simulink model "s_deng_rev1_13_wide"  (R2016b)
(part 3 of 68)

      mask Display:
      | port_label('input', 1, 'd');
      | port_label('output', 1, 'q');
      | disp(['Z^-', num2str(latency)]);
  pipeline80 : Subsystem  AncestorBlock=casper_library_delays/pipeline  mask(pipeline){latency=1}
      mask help:
      | An explicitly laid-out delay line to avoid mapping to SRL16s
      | for use in pipelining to help achieve timing closure.
      mask init:
      | pipeline_init(gcb,'latency',latency);
      settings: AttributesFormatString=Latency = %<latency>
      mask Display:
      | port_label('input', 1, 'd');
      | port_label('output', 1, 'q');
      | disp(['Z^-', num2str(latency)]);
  pipeline81 : Subsystem  AncestorBlock=casper_library_delays/pipeline  mask(pipeline){latency=3}
      mask help:
      | An explicitly laid-out delay line to avoid mapping to SRL16s
      | for use in pipelining to help achieve timing closure.
      mask init:
      | pipeline_init(gcb,'latency',latency);
      settings: AttributesFormatString=Latency = %<latency>
      mask Display:
      | port_label('input', 1, 'd');
      | port_label('output', 1, 'q');
      | disp(['Z^-', num2str(latency)]);
  pipeline82 : Subsystem  AncestorBlock=casper_library_delays/pipeline  mask(pipeline){latency=1}
      mask help:
      | An explicitly laid-out delay line to avoid mapping to SRL16s
      | for use in pipelining to help achieve timing closure.
      mask init:
      | pipeline_init(gcb,'latency',latency);
      settings: AttributesFormatString=Latency = %<latency>
      mask Display:
      | port_label('input', 1, 'd');
      | port_label('output', 1, 'q');
      | disp(['Z^-', num2str(latency)]);
  pipeline83 : Subsystem  AncestorBlock=casper_library_delays/pipeline  mask(pipeline){latency=1}
      mask help:
      | An explicitly laid-out delay line to avoid mapping to SRL16s
      | for use in pipelining to help achieve timing closure.
      mask init:
      | pipeline_init(gcb,'latency',latency);
      settings: AttributesFormatString=Latency = %<latency>
      mask Display:
      | port_label('input', 1, 'd');
      | port_label('output', 1, 'q');
      | disp(['Z^-', num2str(latency)]);
  pipeline84 : Subsystem  AncestorBlock=casper_library_delays/pipeline  mask(pipeline){latency=1}
      mask help:
      | An explicitly laid-out delay line to avoid mapping to SRL16s
      | for use in pipelining to help achieve timing closure.
      mask init:
      | pipeline_init(gcb,'latency',latency);
      settings: AttributesFormatString=Latency = %<latency>
      mask Display:
      | port_label('input', 1, 'd');
      | port_label('output', 1, 'q');
      | disp(['Z^-', num2str(latency)]);
  pipeline85 : Subsystem  AncestorBlock=casper_library_delays/pipeline  mask(pipeline){latency=1}
      mask help:
      | An explicitly laid-out delay line to avoid mapping to SRL16s
      | for use in pipelining to help achieve timing closure.
      mask init:
      | pipeline_init(gcb,'latency',latency);
      settings: AttributesFormatString=Latency = %<latency>
      mask Display:
      | port_label('input', 1, 'd');
      | port_label('output', 1, 'q');
      | disp(['Z^-', num2str(latency)]);
  pipeline86 : Subsystem  AncestorBlock=casper_library_delays/pipeline  mask(pipeline){latency=3}
      mask help:
      | An explicitly laid-out delay line to avoid mapping to SRL16s
      | for use in pipelining to help achieve timing closure.
      mask init:
      | pipeline_init(gcb,'latency',latency);
      settings: AttributesFormatString=Latency = %<latency>
      mask Display:
      | port_label('input', 1, 'd');
      | port_label('output', 1, 'q');
      | disp(['Z^-', num2str(latency)]);
  pipeline87 : Subsystem  AncestorBlock=casper_library_delays/pipeline  mask(pipeline){latency=2}
      mask help:
      | An explicitly laid-out delay line to avoid mapping to SRL16s
      | for use in pipelining to help achieve timing closure.
      mask init:
      | pipeline_init(gcb,'latency',latency);
      settings: AttributesFormatString=Latency = %<latency>
      mask Display:
      | port_label('input', 1, 'd');
      | port_label('output', 1, 'q');
      | disp(['Z^-', num2str(latency)]);
  pipeline88 : Subsystem  AncestorBlock=casper_library_delays/pipeline  mask(pipeline){latency=2}
      mask help:
      | An explicitly laid-out delay line to avoid mapping to SRL16s
      | for use in pipelining to help achieve timing closure.
      mask init:
      | pipeline_init(gcb,'latency',latency);
      settings: AttributesFormatString=Latency = %<latency>
      mask Display:
      | port_label('input', 1, 'd');
      | port_label('output', 1, 'q');
      | disp(['Z^-', num2str(latency)]);
  pipeline89 : Subsystem  AncestorBlock=casper_library_delays/pipeline  mask(pipeline){latency=2}
      mask help:
      | An explicitly laid-out delay line to avoid mapping to SRL16s
      | for use in pipelining to help achieve timing closure.
      mask init:
      | pipeline_init(gcb,'latency',latency);
      settings: AttributesFormatString=Latency = %<latency>
      mask Display:
      | port_label('input', 1, 'd');
      | port_label('output', 1, 'q');
      | disp(['Z^-', num2str(latency)]);
  pipeline9 : Subsystem  AncestorBlock=casper_library_delays/pipeline  mask(pipeline){latency=3}
      mask help:
      | An explicitly laid-out delay line to avoid mapping to SRL16s
      | for use in pipelining to help achieve timing closure.
      mask init:
      | pipeline_init(gcb,'latency',latency);
      settings: AttributesFormatString=Latency = %<latency>
      mask Display:
      | port_label('input', 1, 'd');
      | port_label('output', 1, 'q');
      | disp(['Z^-', num2str(latency)]);
  pipeline90 : Subsystem  AncestorBlock=casper_library_delays/pipeline  mask(pipeline){latency=2}
      mask help:
      | An explicitly laid-out delay line to avoid mapping to SRL16s
      | for use in pipelining to help achieve timing closure.
      mask init:
      | pipeline_init(gcb,'latency',latency);
      settings: AttributesFormatString=Latency = %<latency>
      mask Display:
      | port_label('input', 1, 'd');
      | port_label('output', 1, 'q');
      | disp(['Z^-', num2str(latency)]);
  pipeline91 : Subsystem  AncestorBlock=casper_library_delays/pipeline  mask(pipeline){latency=2}
      mask help:
      | An explicitly laid-out delay line to avoid mapping to SRL16s
      | for use in pipelining to help achieve timing closure.
      mask init:
      | pipeline_init(gcb,'latency',latency);
      settings: AttributesFormatString=Latency = %<latency>
      mask Display:
      | port_label('input', 1, 'd');
      | port_label('output', 1, 'q');
      | disp(['Z^-', num2str(latency)]);
  pipeline92 : Subsystem  AncestorBlock=casper_library_delays/pipeline  mask(pipeline){latency=2}
      mask help:
      | An explicitly laid-out delay line to avoid mapping to SRL16s
      | for use in pipelining to help achieve timing closure.
      mask init:
      | pipeline_init(gcb,'latency',latency);
      settings: AttributesFormatString=Latency = %<latency>
      mask Display:
      | port_label('input', 1, 'd');
      | port_label('output', 1, 'q');
      | disp(['Z^-', num2str(latency)]);
  pipeline93 : Subsystem  AncestorBlock=casper_library_delays/pipeline  mask(pipeline){latency=2}
      mask help:
      | An explicitly laid-out delay line to avoid mapping to SRL16s
      | for use in pipelining to help achieve timing closure.
      mask init:
      | pipeline_init(gcb,'latency',latency);
      settings: AttributesFormatString=Latency = %<latency>
      mask Display:
      | port_label('input', 1, 'd');
      | port_label('output', 1, 'q');
      | disp(['Z^-', num2str(latency)]);
  pipeline94 : Subsystem  AncestorBlock=casper_library_delays/pipeline  mask(pipeline){latency=2}
      mask help:
      | An explicitly laid-out delay line to avoid mapping to SRL16s
      | for use in pipelining to help achieve timing closure.
      mask init:
      | pipeline_init(gcb,'latency',latency);
      settings: AttributesFormatString=Latency = %<latency>
      mask Display:
      | port_label('input', 1, 'd');
      | port_label('output', 1, 'q');
      | disp(['Z^-', num2str(latency)]);
  pipeline95 : Subsystem  AncestorBlock=casper_library_delays/pipeline  mask(pipeline){latency=2}
      mask help:
      | An explicitly laid-out delay line to avoid mapping to SRL16s
      | for use in pipelining to help achieve timing closure.
      mask init:
      | pipeline_init(gcb,'latency',latency);
      settings: AttributesFormatString=Latency = %<latency>
      mask Display:
      | port_label('input', 1, 'd');
      | port_label('output', 1, 'q');
      | disp(['Z^-', num2str(latency)]);
  pipeline96 : Subsystem  AncestorBlock=casper_library_delays/pipeline  mask(pipeline){latency=2}
      mask help:
      | An explicitly laid-out delay line to avoid mapping to SRL16s
      | for use in pipelining to help achieve timing closure.
      mask init:
      | pipeline_init(gcb,'latency',latency);
      settings: AttributesFormatString=Latency = %<latency>
      mask Display:
      | port_label('input', 1, 'd');
      | port_label('output', 1, 'q');
      | disp(['Z^-', num2str(latency)]);
  pipeline97 : Subsystem  AncestorBlock=casper_library_delays/pipeline  mask(pipeline){latency=2}
      mask help:
      | An explicitly laid-out delay line to avoid mapping to SRL16s
      | for use in pipelining to help achieve timing closure.
      mask init:
      | pipeline_init(gcb,'latency',latency);
      settings: AttributesFormatString=Latency = %<latency>
      mask Display:
      | port_label('input', 1, 'd');
      | port_label('output', 1, 'q');
      | disp(['Z^-', num2str(latency)]);
  pipeline98 : Subsystem  AncestorBlock=casper_library_delays/pipeline  mask(pipeline){latency=2}
      mask help:
      | An explicitly laid-out delay line to avoid mapping to SRL16s
      | for use in pipelining to help achieve timing closure.
      mask init:
      | pipeline_init(gcb,'latency',latency);
      settings: AttributesFormatString=Latency = %<latency>
      mask Display:
      | port_label('input', 1, 'd');
      | port_label('output', 1, 'q');
      | disp(['Z^-', num2str(latency)]);
  pipeline99 : Subsystem  AncestorBlock=casper_library_delays/pipeline  mask(pipeline){latency=2}
      mask help:
      | An explicitly laid-out delay line to avoid mapping to SRL16s
      | for use in pipelining to help achieve timing closure.
      mask init:
      | pipeline_init(gcb,'latency',latency);
      settings: AttributesFormatString=Latency = %<latency>
      mask Display:
      | port_label('input', 1, 'd');
      | port_label('output', 1, 'q');
      | disp(['Z^-', num2str(latency)]);
  pkt_rate0 : Subsystem
  pkt_size0 : Subsystem  Tag=xps:sw_reg  AncestorBlock=xps_library/software_register  mask(swreg){io_dir=From Processor, io_delay=0, sample_period=1, names=reg, bitwidths=32, bin_pts=0, arith_types=0, sim_port=on, show_format=on}
      mask prompts: io_dir "I/O direction"; io_delay "I/O delay"; sample_period "Sample period"; names "Bitfield names [msb...lsb]"; bitwidths "Bitfield widths"; bin_pts "Bitfield binary pts"; arith_types "Bitfield types, ufix=0, fix=1, bool=2"; sim_port "Provide sim input/output?"; show_format "Print format string?"
      mask help: A 32-bit software-accessible register. Can be divided into bitfields of varying widths and types using the fields in the block mask.
      mask init:
      | swreg_init(gcb)
      settings: AttributesFormatString=1input:uf32.0 = 32 bits
      mask TypeOptions io_dir: To Processor | From Processor
      mask Callback io_dir:
      | mask_enables = get_param(gcb, 'MaskEnables');
      | mask_names = get_param(gcb, 'MaskNames');
      | if strcmp(get_param(gcb, 'io_dir'), 'To Processor'),
      |     mask_enables{ismember(mask_names, 'sample_period')} = 'off';
      | else
      |     mask_enables{ismember(mask_names, 'sample_period')} = 'on';
      | end
      | set_param(gcb, 'MaskEnables', mask_enables);
  pkt_size_calc0 : Subsystem
  pol0_num_pkts : Subsystem  Tag=xps:sw_reg  AncestorBlock=xps_library/software_register  mask(swreg){io_dir=From Processor, io_delay=1, sample_period=1, names=pol0_num_pkts, bitwidths=32, bin_pts=0, arith_types=0, sim_port=on, show_format=on}
      mask prompts: io_dir "I/O direction"; io_delay "I/O delay"; sample_period "Sample period"; names "Bitfield names [msb...lsb]"; bitwidths "Bitfield widths"; bin_pts "Bitfield binary pts"; arith_types "Bitfield types, ufix=0, fix=1, bool=2"; sim_port "Provide sim input/output?"; show_format "Print format string?"
      mask help: A 32-bit software-accessible register. Can be divided into bitfields of varying widths and types using the fields in the block mask.
      mask init:
      | swreg_init(gcb)
      settings: AttributesFormatString=1input:uf32.0 = 32 bits
      mask TypeOptions io_dir: To Processor | From Processor
      mask Callback io_dir:
      | mask_enables = get_param(gcb, 'MaskEnables');
      | mask_names = get_param(gcb, 'MaskNames');
      | if strcmp(get_param(gcb, 'io_dir'), 'To Processor'),
      |     mask_enables{ismember(mask_names, 'sample_period')} = 'off';
      | else
      |     mask_enables{ismember(mask_names, 'sample_period')} = 'on';
      | end
      | set_param(gcb, 'MaskEnables', mask_enables);
  pol0_sample_offset : Subsystem  Tag=xps:sw_reg  AncestorBlock=xps_library/software_register  mask(swreg){io_dir=From Processor, io_delay=1, sample_period=1, names=pol0_sample_offset, bitwidths=18, bin_pts=0, arith_types=0, sim_port=on, show_format=on}
      mask prompts: io_dir "I/O direction"; io_delay "I/O delay"; sample_period "Sample period"; names "Bitfield names [msb...lsb]"; bitwidths "Bitfield widths"; bin_pts "Bitfield binary pts"; arith_types "Bitfield types, ufix=0, fix=1, bool=2"; sim_port "Provide sim input/output?"; show_format "Print format string?"
      mask help: A 32-bit software-accessible register. Can be divided into bitfields of varying widths and types using the fields in the block mask.
      mask init:
      | swreg_init(gcb)
      settings: AttributesFormatString=1input:uf18.0 = 18 bits
      mask TypeOptions io_dir: To Processor | From Processor
      mask Callback io_dir:
      | mask_enables = get_param(gcb, 'MaskEnables');
      | mask_names = get_param(gcb, 'MaskNames');
      | if strcmp(get_param(gcb, 'io_dir'), 'To Processor'),
      |     mask_enables{ismember(mask_names, 'sample_period')} = 'off';
      | else
      |     mask_enables{ismember(mask_names, 'sample_period')} = 'on';
      | end
      | set_param(gcb, 'MaskEnables', mask_enables);
  pol1_num_pkts : Subsystem  Tag=xps:sw_reg  AncestorBlock=xps_library/software_register  mask(swreg){io_dir=From Processor, io_delay=1, sample_period=1, names=pol1_num_pkts, bitwidths=32, bin_pts=0, arith_types=0, sim_port=on, show_format=on}
      mask prompts: io_dir "I/O direction"; io_delay "I/O delay"; sample_period "Sample period"; names "Bitfield names [msb...lsb]"; bitwidths "Bitfield widths"; bin_pts "Bitfield binary pts"; arith_types "Bitfield types, ufix=0, fix=1, bool=2"; sim_port "Provide sim input/output?"; show_format "Print format string?"
      mask help: A 32-bit software-accessible register. Can be divided into bitfields of varying widths and types using the fields in the block mask.
      mask init:
      | swreg_init(gcb)
      settings: AttributesFormatString=1input:uf32.0 = 32 bits
      mask TypeOptions io_dir: To Processor | From Processor
      mask Callback io_dir:
      | mask_enables = get_param(gcb, 'MaskEnables');
      | mask_names = get_param(gcb, 'MaskNames');
      | if strcmp(get_param(gcb, 'io_dir'), 'To Processor'),
      |     mask_enables{ismember(mask_names, 'sample_period')} = 'off';
      | else
      |     mask_enables{ismember(mask_names, 'sample_period')} = 'on';
      | end
      | set_param(gcb, 'MaskEnables', mask_enables);
  pol1_sample_offset : Subsystem  Tag=xps:sw_reg  AncestorBlock=xps_library/software_register  mask(swreg){io_dir=From Processor, io_delay=1, sample_period=1, names=pol1_sample_offset, bitwidths=18, bin_pts=0, arith_types=0, sim_port=on, show_format=on}
      mask prompts: io_dir "I/O direction"; io_delay "I/O delay"; sample_period "Sample period"; names "Bitfield names [msb...lsb]"; bitwidths "Bitfield widths"; bin_pts "Bitfield binary pts"; arith_types "Bitfield types, ufix=0, fix=1, bool=2"; sim_port "Provide sim input/output?"; show_format "Print format string?"
      mask help: A 32-bit software-accessible register. Can be divided into bitfields of varying widths and types using the fields in the block mask.
      mask init:
      | swreg_init(gcb)
      settings: AttributesFormatString=1input:uf18.0 = 18 bits
      mask TypeOptions io_dir: To Processor | From Processor
      mask Callback io_dir:
      | mask_enables = get_param(gcb, 'MaskEnables');
      | mask_names = get_param(gcb, 'MaskNames');
      | if strcmp(get_param(gcb, 'io_dir'), 'To Processor'),
      |     mask_enables{ismember(mask_names, 'sample_period')} = 'off';
      | else
      |     mask_enables{ismember(mask_names, 'sample_period')} = 'on';
      | end
      | set_param(gcb, 'MaskEnables', mask_enables);
  pol_traffic_trigger : Subsystem  Tag=xps:sw_reg  AncestorBlock=xps_library/software_register  mask(swreg){io_dir=From Processor, io_delay=1, sample_period=1, names=[pol0_tx_trigger pol1_tx_trigger], bitwidths=[1 1], bin_pts=[0 0], arith_types=[2 2], sim_port=on, show_format=on}
      mask prompts: io_dir "I/O direction"; io_delay "I/O delay"; sample_period "Sample period"; names "Bitfield names [msb...lsb]"; bitwidths "Bitfield widths"; bin_pts "Bitfield binary pts"; arith_types "Bitfield types, ufix=0, fix=1, bool=2"; sim_port "Provide sim input/output?"; show_format "Print format string?"
      mask help: A 32-bit software-accessible register. Can be divided into bitfields of varying widths and types using the fields in the block mask.
      mask init:
      | swreg_init(gcb)
      settings: AttributesFormatString=2 inputs:b,b = 2 bits
      mask TypeOptions io_dir: To Processor | From Processor
      mask Callback io_dir:
      | mask_enables = get_param(gcb, 'MaskEnables');
      | mask_names = get_param(gcb, 'MaskNames');
      | if strcmp(get_param(gcb, 'io_dir'), 'To Processor'),
      |     mask_enables{ismember(mask_names, 'sample_period')} = 'off';
      | else
      |     mask_enables{ismember(mask_names, 'sample_period')} = 'on';
      | end
      | set_param(gcb, 'MaskEnables', mask_enables);
  pol_tx_always_on : Subsystem  Tag=xps:sw_reg  AncestorBlock=xps_library/software_register  mask(swreg){io_dir=From Processor, io_delay=1, sample_period=1, names=[pol0_tx_always_on pol1_tx_always_on], bitwidths=[1 1], bin_pts=[0 0], arith_types=[2 2], sim_port=on, show_format=on}
      mask prompts: io_dir "I/O direction"; io_delay "I/O delay"; sample_period "Sample period"; names "Bitfield names [msb...lsb]"; bitwidths "Bitfield widths"; bin_pts "Bitfield binary pts"; arith_types "Bitfield types, ufix=0, fix=1, bool=2"; sim_port "Provide sim input/output?"; show_format "Print format string?"
      mask help: A 32-bit software-accessible register. Can be divided into bitfields of varying widths and types using the fields in the block mask.
      mask init:
      | swreg_init(gcb)
      settings: AttributesFormatString=2 inputs:b,b = 2 bits
      mask TypeOptions io_dir: To Processor | From Processor
      mask Callback io_dir:
      | mask_enables = get_param(gcb, 'MaskEnables');
      | mask_names = get_param(gcb, 'MaskNames');
      | if strcmp(get_param(gcb, 'io_dir'), 'To Processor'),
      |     mask_enables{ismember(mask_names, 'sample_period')} = 'off';
      | else
      |     mask_enables{ismember(mask_names, 'sample_period')} = 'on';
      | end
      | set_param(gcb, 'MaskEnables', mask_enables);
      mask DialogControl ParameterTabVar0 Prompt: Setup
  ramp{0..3} (4 alike) : xbsIndex_r4/Counter  cnt_type=Free Running  cnt_to=Inf  operation=Up  start_count=0  cnt_by_val=1  arith_type=Unsigned  n_bits=64  bin_pt=0  load_pin=off  rst=on  en=on  explicit_period=on  period=1  use_behavioral_HDL=off  implementation=Fabric  dbl_ovrd=off  block_type=counter
  ramp80 : xbsIndex_r4/Counter  cnt_type=Free Running  cnt_to=Inf  operation=Up  start_count=0  cnt_by_val=1  arith_type=Unsigned  n_bits=79  bin_pt=0  load_pin=off  rst=on  en=off  explicit_period=on  period=1  use_behavioral_HDL=off  implementation=Fabric  dbl_ovrd=off  block_type=counter
  ramp_control : Subsystem  Tag=xps:sw_reg  AncestorBlock=xps_library/software_register  mask(swreg){io_dir=From Processor, io_delay=0, sample_period=1, names=[sel_ramp80 rst_ramp80 sel_munge sel_insert_time], bitwidths=1, bin_pts=0, arith_types=2, sim_port=on, show_format=on}
      mask prompts: io_dir "I/O direction"; io_delay "I/O delay"; sample_period "Sample period"; names "Bitfield names [msb...lsb]"; bitwidths "Bitfield widths"; bin_pts "Bitfield binary pts"; arith_types "Bitfield types, ufix=0, fix=1, bool=2"; sim_port "Provide sim input/output?"; show_format "Print format string?"
      mask help: A 32-bit software-accessible register. Can be divided into bitfields of varying widths and types using the fields in the block mask.
      mask init:
      | swreg_init(gcb)
      settings: AttributesFormatString=4 inputs:b,b,b,b = 4 bits
      mask TypeOptions io_dir: To Processor | From Processor
      mask Callback io_dir:
      | mask_enables = get_param(gcb, 'MaskEnables');
      | mask_names = get_param(gcb, 'MaskNames');
      | if strcmp(get_param(gcb, 'io_dir'), 'To Processor'),
      |     mask_enables{ismember(mask_names, 'sample_period')} = 'off';
      | else
      |     mask_enables{ismember(mask_names, 'sample_period')} = 'on';
      | end
      | set_param(gcb, 'MaskEnables', mask_enables);
  rd_addr{0..3} (4 alike) : xbsIndex_r4/Counter  cnt_type=Free Running  cnt_to=Inf  operation=Up  start_count=0  cnt_by_val=1  arith_type=Unsigned  n_bits=8  bin_pt=0  load_pin=off  rst=on  en=on  explicit_period=on  period=1  use_behavioral_HDL=off  implementation=Fabric  dbl_ovrd=off  block_type=counter
  rd_arm{,1..3} (4 alike) : xbsIndex_r4/Register  init=0  rst=on  en=on  dbl_ovrd=off  block_type=register
  receptor_id : Subsystem  Tag=xps:sw_reg  AncestorBlock=xps_library/software_register  mask(swreg){io_dir=From Processor, io_delay=1, sample_period=1, names=[receptor_id pol0_id pol1_id], bitwidths=[14 2 2], bin_pts=[0 0 0], arith_types=[0 0 0], sim_port=on, show_format=on}
      mask prompts: io_dir "I/O direction"; io_delay "I/O delay"; sample_period "Sample period"; names "Bitfield names [msb...lsb]"; bitwidths "Bitfield widths"; bin_pts "Bitfield binary pts"; arith_types "Bitfield types, ufix=0, fix=1, bool=2"; sim_port "Provide sim input/output?"; show_format "Print format string?"
      mask help: A 32-bit software-accessible register. Can be divided into bitfields of varying widths and types using the fields in the block mask.
      mask init:
      | swreg_init(gcb)
      settings: AttributesFormatString=3 inputs:uf14.0,uf2.0,uf2.0 = 18 bits
      mask TypeOptions io_dir: To Processor | From Processor
      mask Callback io_dir:
      | mask_enables = get_param(gcb, 'MaskEnables');
      | mask_names = get_param(gcb, 'MaskNames');
      | if strcmp(get_param(gcb, 'io_dir'), 'To Processor'),
      |     mask_enables{ismember(mask_names, 'sample_period')} = 'off';
      | else
      |     mask_enables{ismember(mask_names, 'sample_period')} = 'on';
      | end
      | set_param(gcb, 'MaskEnables', mask_enables);
  rpt_en_cwg0 : Subsystem  Tag=xps:sw_reg  AncestorBlock=xps_library/software_register  mask(swreg){io_dir=From Processor, io_delay=1, sample_period=1, names=en, bitwidths=1, bin_pts=0, arith_types=2, sim_port=on, show_format=on}
      mask prompts: io_dir "I/O direction"; io_delay "I/O delay"; sample_period "Sample period"; names "Bitfield names [msb...lsb]"; bitwidths "Bitfield widths"; bin_pts "Bitfield binary pts"; arith_types "Bitfield types, ufix=0, fix=1, bool=2"; sim_port "Provide sim input/output?"; show_format "Print format string?"
      mask help: A 32-bit software-accessible register. Can be divided into bitfields of varying widths and types using the fields in the block mask.
      mask init:
      | swreg_init(gcb)
      settings: AttributesFormatString=1input:b = 1 bits
      mask TypeOptions io_dir: To Processor | From Processor
      mask Callback io_dir:
      | mask_enables = get_param(gcb, 'MaskEnables');
      | mask_names = get_param(gcb, 'MaskNames');
      | if strcmp(get_param(gcb, 'io_dir'), 'To Processor'),
      |     mask_enables{ismember(mask_names, 'sample_period')} = 'off';
      | else
      |     mask_enables{ismember(mask_names, 'sample_period')} = 'on';
      | end
      | set_param(gcb, 'MaskEnables', mask_enables);
  rpt_en_cwg1 : Subsystem  Tag=xps:sw_reg  AncestorBlock=xps_library/software_register  mask(swreg){io_dir=From Processor, io_delay=1, sample_period=1, names=en, bitwidths=1, bin_pts=0, arith_types=2, sim_port=on, show_format=on}
      mask prompts: io_dir "I/O direction"; io_delay "I/O delay"; sample_period "Sample period"; names "Bitfield names [msb...lsb]"; bitwidths "Bitfield widths"; bin_pts "Bitfield binary pts"; arith_types "Bitfield types, ufix=0, fix=1, bool=2"; sim_port "Provide sim input/output?"; show_format "Print format string?"
      mask help: A 32-bit software-accessible register. Can be divided into bitfields of varying widths and types using the fields in the block mask.
      mask init:
      | swreg_init(gcb)
      settings: AttributesFormatString=1input:b = 1 bits
      mask TypeOptions io_dir: To Processor | From Processor
      mask Callback io_dir:
      | mask_enables = get_param(gcb, 'MaskEnables');
      | mask_names = get_param(gcb, 'MaskNames');
      | if strcmp(get_param(gcb, 'io_dir'), 'To Processor'),
      |     mask_enables{ismember(mask_names, 'sample_period')} = 'off';
      | else
      |     mask_enables{ismember(mask_names, 'sample_period')} = 'on';
      | end
      | set_param(gcb, 'MaskEnables', mask_enables);
  rpt_en_cwg_corr : Subsystem  Tag=xps:sw_reg  AncestorBlock=xps_library/software_register  mask(swreg){io_dir=From Processor, io_delay=1, sample_period=1, names=en, bitwidths=1, bin_pts=0, arith_types=2, sim_port=on, show_format=on}
      mask prompts: io_dir "I/O direction"; io_delay "I/O delay"; sample_period "Sample period"; names "Bitfield names [msb...lsb]"; bitwidths "Bitfield widths"; bin_pts "Bitfield binary pts"; arith_types "Bitfield types, ufix=0, fix=1, bool=2"; sim_port "Provide sim input/output?"; show_format "Print format string?"
      mask help: A 32-bit software-accessible register. Can be divided into bitfields of varying widths and types using the fields in the block mask.
      mask init:
      | swreg_init(gcb)
      settings: AttributesFormatString=1input:b = 1 bits
      mask TypeOptions io_dir: To Processor | From Processor
      mask Callback io_dir:
      | mask_enables = get_param(gcb, 'MaskEnables');
      | mask_names = get_param(gcb, 'MaskNames');
      | if strcmp(get_param(gcb, 'io_dir'), 'To Processor'),
      |     mask_enables{ismember(mask_names, 'sample_period')} = 'off';
      | else
      |     mask_enables{ismember(mask_names, 'sample_period')} = 'on';
      | end
      | set_param(gcb, 'MaskEnables', mask_enables);
  rpt_length_cwg0 : Subsystem  Tag=xps:sw_reg  AncestorBlock=xps_library/software_register  mask(swreg){io_dir=From Processor, io_delay=1, sample_period=1, names=repeat_length, bitwidths=32, bin_pts=0, arith_types=0, sim_port=on, show_format=on}
      mask prompts: io_dir "I/O direction"; io_delay "I/O delay"; sample_period "Sample period"; names "Bitfield names [msb...lsb]"; bitwidths "Bitfield widths"; bin_pts "Bitfield binary pts"; arith_types "Bitfield types, ufix=0, fix=1, bool=2"; sim_port "Provide sim input/output?"; show_format "Print format string?"
      mask help: A 32-bit software-accessible register. Can be divided into bitfields of varying widths and types using the fields in the block mask.
      mask init:
      | swreg_init(gcb)
      settings: AttributesFormatString=1input:uf32.0 = 32 bits
      mask TypeOptions io_dir: To Processor | From Processor
      mask Callback io_dir:
      | mask_enables = get_param(gcb, 'MaskEnables');
      | mask_names = get_param(gcb, 'MaskNames');
      | if strcmp(get_param(gcb, 'io_dir'), 'To Processor'),
      |     mask_enables{ismember(mask_names, 'sample_period')} = 'off';
      | else
      |     mask_enables{ismember(mask_names, 'sample_period')} = 'on';
      | end
      | set_param(gcb, 'MaskEnables', mask_enables);
  rpt_length_cwg1 : Subsystem  Tag=xps:sw_reg  AncestorBlock=xps_library/software_register  mask(swreg){io_dir=From Processor, io_delay=1, sample_period=1, names=repeat_length, bitwidths=32, bin_pts=0, arith_types=0, sim_port=on, show_format=on}
      mask prompts: io_dir "I/O direction"; io_delay "I/O delay"; sample_period "Sample period"; names "Bitfield names [msb...lsb]"; bitwidths "Bitfield widths"; bin_pts "Bitfield binary pts"; arith_types "Bitfield types, ufix=0, fix=1, bool=2"; sim_port "Provide sim input/output?"; show_format "Print format string?"
      mask help: A 32-bit software-accessible register. Can be divided into bitfields of varying widths and types using the fields in the block mask.
      mask init:
      | swreg_init(gcb)
      settings: AttributesFormatString=1input:uf32.0 = 32 bits
      mask TypeOptions io_dir: To Processor | From Processor
      mask Callback io_dir:
      | mask_enables = get_param(gcb, 'MaskEnables');
      | mask_names = get_param(gcb, 'MaskNames');
      | if strcmp(get_param(gcb, 'io_dir'), 'To Processor'),
      |     mask_enables{ismember(mask_names, 'sample_period')} = 'off';
      | else
      |     mask_enables{ismember(mask_names, 'sample_period')} = 'on';
      | end
      | set_param(gcb, 'MaskEnables', mask_enables);
  rpt_length_cwg_corr : Subsystem  Tag=xps:sw_reg  AncestorBlock=xps_library/software_register  mask(swreg){io_dir=From Processor, io_delay=1, sample_period=1, names=repeat_length, bitwidths=32, bin_pts=0, arith_types=0, sim_port=on, show_format=on}
      mask prompts: io_dir "I/O direction"; io_delay "I/O delay"; sample_period "Sample period"; names "Bitfield names [msb...lsb]"; bitwidths "Bitfield widths"; bin_pts "Bitfield binary pts"; arith_types "Bitfield types, ufix=0, fix=1, bool=2"; sim_port "Provide sim input/output?"; show_format "Print format string?"
      mask help: A 32-bit software-accessible register. Can be divided into bitfields of varying widths and types using the fields in the block mask.
      mask init:
      | swreg_init(gcb)
      settings: AttributesFormatString=1input:uf32.0 = 32 bits
      mask TypeOptions io_dir: To Processor | From Processor
      mask Callback io_dir:
      | mask_enables = get_param(gcb, 'MaskEnables');
      | mask_names = get_param(gcb, 'MaskNames');
      | if strcmp(get_param(gcb, 'io_dir'), 'To Processor'),
      |     mask_enables{ismember(mask_names, 'sample_period')} = 'off';
      | else
      |     mask_enables{ismember(mask_names, 'sample_period')} = 'on';
      | end
      | set_param(gcb, 'MaskEnables', mask_enables);
  rpt_length_wng0 : Subsystem  Tag=xps:sw_reg  AncestorBlock=xps_library/software_register  mask(swreg){io_dir=From Processor, io_delay=1, sample_period=1, names=samples, bitwidths=32, bin_pts=0, arith_types=0, sim_port=on, show_format=on}
      mask prompts: io_dir "I/O direction"; io_delay "I/O delay"; sample_period "Sample period"; names "Bitfield names [msb...lsb]"; bitwidths "Bitfield widths"; bin_pts "Bitfield binary pts"; arith_types "Bitfield types, ufix=0, fix=1, bool=2"; sim_port "Provide sim input/output?"; show_format "Print format string?"
      mask help: A 32-bit software-accessible register. Can be divided into bitfields of varying widths and types using the fields in the block mask.
      mask init:
      | swreg_init(gcb)
      settings: AttributesFormatString=1input:uf32.0 = 32 bits
      mask TypeOptions io_dir: To Processor | From Processor
      mask Callback io_dir:
      | mask_enables = get_param(gcb, 'MaskEnables');
      | mask_names = get_param(gcb, 'MaskNames');
      | if strcmp(get_param(gcb, 'io_dir'), 'To Processor'),
      |     mask_enables{ismember(mask_names, 'sample_period')} = 'off';
      | else
      |     mask_enables{ismember(mask_names, 'sample_period')} = 'on';
      | end
      | set_param(gcb, 'MaskEnables', mask_enables);
  rpt_load_time_lsw_wng0 : Subsystem  Tag=xps:sw_reg  AncestorBlock=xps_library/software_register  mask(swreg){io_dir=From Processor, io_delay=1, sample_period=1, names=reg, bitwidths=32, bin_pts=0, arith_types=0, sim_port=on, show_format=on}
      mask prompts: io_dir "I/O direction"; io_delay "I/O delay"; sample_period "Sample period"; names "Bitfield names [msb...lsb]"; bitwidths "Bitfield widths"; bin_pts "Bitfield binary pts"; arith_types "Bitfield types, ufix=0, fix=1, bool=2"; sim_port "Provide sim input/output?"; show_format "Print format string?"
      mask help: A 32-bit software-accessible register. Can be divided into bitfields of varying widths and types using the fields in the block mask.
      mask init:
      | swreg_init(gcb)
      settings: AttributesFormatString=1input:uf32.0 = 32 bits
      mask TypeOptions io_dir: To Processor | From Processor
      mask Callback io_dir:
      | mask_enables = get_param(gcb, 'MaskEnables');
      | mask_names = get_param(gcb, 'MaskNames');
      | if strcmp(get_param(gcb, 'io_dir'), 'To Processor'),
      |     mask_enables{ismember(mask_names, 'sample_period')} = 'off';
      | else
      |     mask_enables{ismember(mask_names, 'sample_period')} = 'on';
      | end
      | set_param(gcb, 'MaskEnables', mask_enables);
  rpt_load_time_msw_wng0 : Subsystem  Tag=xps:sw_reg  AncestorBlock=xps_library/software_register  mask(swreg){io_dir=From Processor, io_delay=1, sample_period=1, names=reg, bitwidths=32, bin_pts=0, arith_types=0, sim_port=on, show_format=on}
      mask prompts: io_dir "I/O direction"; io_delay "I/O delay"; sample_period "Sample period"; names "Bitfield names [msb...lsb]"; bitwidths "Bitfield widths"; bin_pts "Bitfield binary pts"; arith_types "Bitfield types, ufix=0, fix=1, bool=2"; sim_port "Provide sim input/output?"; show_format "Print format string?"
      mask help: A 32-bit software-accessible register. Can be divided into bitfields of varying widths and types using the fields in the block mask.
      mask init:
      | swreg_init(gcb)
      settings: AttributesFormatString=1input:uf32.0 = 32 bits
      mask TypeOptions io_dir: To Processor | From Processor
      mask Callback io_dir:
      | mask_enables = get_param(gcb, 'MaskEnables');
      | mask_names = get_param(gcb, 'MaskNames');
      | if strcmp(get_param(gcb, 'io_dir'), 'To Processor'),
      |     mask_enables{ismember(mask_names, 'sample_period')} = 'off';
      | else
      |     mask_enables{ismember(mask_names, 'sample_period')} = 'on';
      | end
      | set_param(gcb, 'MaskEnables', mask_enables);
  sample_masking : Subsystem  mask{dbwidth=1}
      mask prompts: dbwidth "Data bitwidth:"
  scale_cwg0 : Subsystem  Tag=xps:sw_reg  AncestorBlock=xps_library/software_register  mask(swreg){io_dir=From Processor, io_delay=1, sample_period=1, names=scale, bitwidths=16, bin_pts=15, arith_types=0, sim_port=on, show_format=on}
      mask prompts: io_dir "I/O direction"; io_delay "I/O delay"; sample_period "Sample period"; names "Bitfield names [msb...lsb]"; bitwidths "Bitfield widths"; bin_pts "Bitfield binary pts"; arith_types "Bitfield types, ufix=0, fix=1, bool=2"; sim_port "Provide sim input/output?"; show_format "Print format string?"
      mask help: A 32-bit software-accessible register. Can be divided into bitfields of varying widths and types using the fields in the block mask.
      mask init:
      | swreg_init(gcb)
      settings: AttributesFormatString=1input:uf16.15 = 16 bits
      mask TypeOptions io_dir: To Processor | From Processor
      mask Callback io_dir:
      | mask_enables = get_param(gcb, 'MaskEnables');
      | mask_names = get_param(gcb, 'MaskNames');
      | if strcmp(get_param(gcb, 'io_dir'), 'To Processor'),
      |     mask_enables{ismember(mask_names, 'sample_period')} = 'off';
      | else
      |     mask_enables{ismember(mask_names, 'sample_period')} = 'on';
      | end
      | set_param(gcb, 'MaskEnables', mask_enables);
  scale_cwg1 : Subsystem  Tag=xps:sw_reg  AncestorBlock=xps_library/software_register  mask(swreg){io_dir=From Processor, io_delay=1, sample_period=1, names=scale, bitwidths=16, bin_pts=15, arith_types=0, sim_port=on, show_format=on}
      mask prompts: io_dir "I/O direction"; io_delay "I/O delay"; sample_period "Sample period"; names "Bitfield names [msb...lsb]"; bitwidths "Bitfield widths"; bin_pts "Bitfield binary pts"; arith_types "Bitfield types, ufix=0, fix=1, bool=2"; sim_port "Provide sim input/output?"; show_format "Print format string?"
      mask help: A 32-bit software-accessible register. Can be divided into bitfields of varying widths and types using the fields in the block mask.
      mask init:
      | swreg_init(gcb)
      settings: AttributesFormatString=1input:uf16.15 = 16 bits
      mask TypeOptions io_dir: To Processor | From Processor
      mask Callback io_dir:
      | mask_enables = get_param(gcb, 'MaskEnables');
      | mask_names = get_param(gcb, 'MaskNames');
      | if strcmp(get_param(gcb, 'io_dir'), 'To Processor'),
      |     mask_enables{ismember(mask_names, 'sample_period')} = 'off';
      | else
      |     mask_enables{ismember(mask_names, 'sample_period')} = 'on';
      | end
      | set_param(gcb, 'MaskEnables', mask_enables);
  scale_cwg_corr : Subsystem  Tag=xps:sw_reg  AncestorBlock=xps_library/software_register  mask(swreg){io_dir=From Processor, io_delay=1, sample_period=1, names=scale, bitwidths=16, bin_pts=15, arith_types=0, sim_port=on, show_format=on}
      mask prompts: io_dir "I/O direction"; io_delay "I/O delay"; sample_period "Sample period"; names "Bitfield names [msb...lsb]"; bitwidths "Bitfield widths"; bin_pts "Bitfield binary pts"; arith_types "Bitfield types, ufix=0, fix=1, bool=2"; sim_port "Provide sim input/output?"; show_format "Print format string?"
      mask help: A 32-bit software-accessible register. Can be divided into bitfields of varying widths and types using the fields in the block mask.
      mask init:
      | swreg_init(gcb)
      settings: AttributesFormatString=1input:uf16.15 = 16 bits
      mask TypeOptions io_dir: To Processor | From Processor
      mask Callback io_dir:
      | mask_enables = get_param(gcb, 'MaskEnables');
      | mask_names = get_param(gcb, 'MaskNames');
      | if strcmp(get_param(gcb, 'io_dir'), 'To Processor'),
      |     mask_enables{ismember(mask_names, 'sample_period')} = 'off';
      | else
      |     mask_enables{ismember(mask_names, 'sample_period')} = 'on';
      | end
      | set_param(gcb, 'MaskEnables', mask_enables);
  scale_out0 : Subsystem  Tag=xps:sw_reg  AncestorBlock=xps_library/software_register  mask(swreg){io_dir=From Processor, io_delay=1, sample_period=1, names=scale, bitwidths=16, bin_pts=15, arith_types=0, sim_port=on, show_format=on}
      mask prompts: io_dir "I/O direction"; io_delay "I/O delay"; sample_period "Sample period"; names "Bitfield names [msb...lsb]"; bitwidths "Bitfield widths"; bin_pts "Bitfield binary pts"; arith_types "Bitfield types, ufix=0, fix=1, bool=2"; sim_port "Provide sim input/output?"; show_format "Print format string?"
      mask help: A 32-bit software-accessible register. Can be divided into bitfields of varying widths and types using the fields in the block mask.
      mask init:
      | swreg_init(gcb)
      settings: AttributesFormatString=1input:uf16.15 = 16 bits
      mask TypeOptions io_dir: To Processor | From Processor
      mask Callback io_dir:
      | mask_enables = get_param(gcb, 'MaskEnables');
      | mask_names = get_param(gcb, 'MaskNames');
      | if strcmp(get_param(gcb, 'io_dir'), 'To Processor'),
      |     mask_enables{ismember(mask_names, 'sample_period')} = 'off';
      | else
      |     mask_enables{ismember(mask_names, 'sample_period')} = 'on';
      | end
      | set_param(gcb, 'MaskEnables', mask_enables);
  scale_out1 : Subsystem  Tag=xps:sw_reg  AncestorBlock=xps_library/software_register  mask(swreg){io_dir=From Processor, io_delay=1, sample_period=1, names=scale, bitwidths=16, bin_pts=15, arith_types=0, sim_port=on, show_format=on}
      mask prompts: io_dir "I/O direction"; io_delay "I/O delay"; sample_period "Sample period"; names "Bitfield names [msb...lsb]"; bitwidths "Bitfield widths"; bin_pts "Bitfield binary pts"; arith_types "Bitfield types, ufix=0, fix=1, bool=2"; sim_port "Provide sim input/output?"; show_format "Print format string?"
      mask help: A 32-bit software-accessible register. Can be divided into bitfields of varying widths and types using the fields in the block mask.
      mask init:
      | swreg_init(gcb)
      settings: AttributesFormatString=1input:uf16.15 = 16 bits
      mask TypeOptions io_dir: To Processor | From Processor
      mask Callback io_dir:
      | mask_enables = get_param(gcb, 'MaskEnables');
      | mask_names = get_param(gcb, 'MaskNames');
      | if strcmp(get_param(gcb, 'io_dir'), 'To Processor'),
      |     mask_enables{ismember(mask_names, 'sample_period')} = 'off';
      | else
      |     mask_enables{ismember(mask_names, 'sample_period')} = 'on';
      | end
      | set_param(gcb, 'MaskEnables', mask_enables);
  scale_wng0 : Subsystem  Tag=xps:sw_reg  AncestorBlock=xps_library/software_register  mask(swreg){io_dir=From Processor, io_delay=1, sample_period=1, names=scale, bitwidths=16, bin_pts=15, arith_types=0, sim_port=on, show_format=on}
      mask prompts: io_dir "I/O direction"; io_delay "I/O delay"; sample_period "Sample period"; names "Bitfield names [msb...lsb]"; bitwidths "Bitfield widths"; bin_pts "Bitfield binary pts"; arith_types "Bitfield types, ufix=0, fix=1, bool=2"; sim_port "Provide sim input/output?"; show_format "Print format string?"
      mask help: A 32-bit software-accessible register. Can be divided into bitfields of varying widths and types using the fields in the block mask.
      mask init:
      | swreg_init(gcb)
      settings: AttributesFormatString=1input:uf16.15 = 16 bits
      mask TypeOptions io_dir: To Processor | From Processor
      mask Callback io_dir:
      | mask_enables = get_param(gcb, 'MaskEnables');
      | mask_names = get_param(gcb, 'MaskNames');
      | if strcmp(get_param(gcb, 'io_dir'), 'To Processor'),
      |     mask_enables{ismember(mask_names, 'sample_period')} = 'off';
      | else
      |     mask_enables{ismember(mask_names, 'sample_period')} = 'on';
      | end
      | set_param(gcb, 'MaskEnables', mask_enables);
  scale_wng1 : Subsystem  Tag=xps:sw_reg  AncestorBlock=xps_library/software_register  mask(swreg){io_dir=From Processor, io_delay=1, sample_period=1, names=scale, bitwidths=16, bin_pts=15, arith_types=0, sim_port=on, show_format=on}
      mask prompts: io_dir "I/O direction"; io_delay "I/O delay"; sample_period "Sample period"; names "Bitfield names [msb...lsb]"; bitwidths "Bitfield widths"; bin_pts "Bitfield binary pts"; arith_types "Bitfield types, ufix=0, fix=1, bool=2"; sim_port "Provide sim input/output?"; show_format "Print format string?"
      mask help: A 32-bit software-accessible register. Can be divided into bitfields of varying widths and types using the fields in the block mask.
      mask init:
      | swreg_init(gcb)
      settings: AttributesFormatString=1input:uf16.15 = 16 bits
      mask TypeOptions io_dir: To Processor | From Processor
      mask Callback io_dir:
      | mask_enables = get_param(gcb, 'MaskEnables');
      | mask_names = get_param(gcb, 'MaskNames');
      | if strcmp(get_param(gcb, 'io_dir'), 'To Processor'),
      |     mask_enables{ismember(mask_names, 'sample_period')} = 'off';
      | else
      |     mask_enables{ismember(mask_names, 'sample_period')} = 'on';
      | end
      | set_param(gcb, 'MaskEnables', mask_enables);
  scale_wng_corr : Subsystem  Tag=xps:sw_reg  AncestorBlock=xps_library/software_register  mask(swreg){io_dir=From Processor, io_delay=1, sample_period=1, names=scale, bitwidths=16, bin_pts=15, arith_types=0, sim_port=on, show_format=on}
      mask prompts: io_dir "I/O direction"; io_delay "I/O delay"; sample_period "Sample period"; names "Bitfield names [msb...lsb]"; bitwidths "Bitfield widths"; bin_pts "Bitfield binary pts"; arith_types "Bitfield types, ufix=0, fix=1, bool=2"; sim_port "Provide sim input/output?"; show_format "Print format string?"
      mask help: A 32-bit software-accessible register. Can be divided into bitfields of varying widths and types using the fields in the block mask.
      mask init:
      | swreg_init(gcb)
      settings: AttributesFormatString=1input:uf16.15 = 16 bits
      mask TypeOptions io_dir: To Processor | From Processor
      mask Callback io_dir:
      | mask_enables = get_param(gcb, 'MaskEnables');
      | mask_names = get_param(gcb, 'MaskNames');
      | if strcmp(get_param(gcb, 'io_dir'), 'To Processor'),
      |     mask_enables{ismember(mask_names, 'sample_period')} = 'off';
      | else
      |     mask_enables{ismember(mask_names, 'sample_period')} = 'on';
      | end
      | set_param(gcb, 'MaskEnables', mask_enables);
  slice1 : xbsIndex_r4/Slice  nbits=32  boolean_output=off  mode=Lower Bit Location + Width  bit1=-7  base1=MSB of Input  bit0=0  base0=LSB of Input  dbl_ovrd=off  block_type=slice
  slice2 : xbsIndex_r4/Slice  nbits=32  boolean_output=off  mode=Lower Bit Location + Width  bit1=-32  base1=MSB of Input  bit0=32  base0=LSB of Input  dbl_ovrd=off  block_type=slice
  spead_detail : Subsystem  Tag=casper:bitsnap  AncestorBlock=casper_library_scopes/bitfield_snapshot  mask(bitsnap){io_names=[eof we], io_widths=1, io_bps=0, io_types=2, show_format=on, snap_storage=bram, snap_dram_dimm=2, snap_dram_clock=250, snap_nsamples=15, snap_data_width=32, snap_offset=off, snap_circap=off, snap_value=off, snap_ext_arm=off, snap_ext_circ=off, snap_provide_outputs=on, snap_use_dsp48=on, snap_delay=2, extra_names=[c d], extra_widths=[30 2], extra_bps=[0 0], extra_types=[0 0]}
      mask prompts: io_names "Names [msb...lsb]"; io_widths "Bitwidths [msb...lsb]"; io_bps "Binary pts [msb...lsb]"; io_types "Data types [msb...lsb], ufix=0, fix=1, bool=2"; show_format "Print format string?"; snap_storage "Storage medium"; snap_dram_dimm "DRAM dimm"; snap_dram_clock "DRAM clock rate"; snap_nsamples "Number of Samples (2^?)"; snap_data_width "Data width"; snap_offset "Start delay support"; snap_circap "Circular capture support"; snap_value "Extra value capture support"; snap_ext_arm "External arm support"; snap_ext_circ "External circular capture support"; snap_provide_outputs "Provide outputs"; snap_use_dsp48 "Use DSP48s to implement counters"; snap_delay "Pre-snapshot delay"; extra_names "Names [msb...lsb]"; extra_widths "Widths [msb...lsb]"; extra_bps "Binary pts [msb...lsb]"; extra_types "Data types [msb...lsb], ufix=0, fix=1, bool=2"
      mask help:
      | A wrapped snapshot block. Allows specification of inputs to a snapblock word so the toolflow can automatically set up the scope.
      | See documentation for snapshot for explanation of parameters.
      mask init:
      | bitsnap_init(gcb);
      settings: AttributesFormatString=|
      | snap(2):b,b = 2 bits\n32 wide, 32768 deep
      | debugID: 29988897
      mask TypeOptions snap_storage: bram | dram
      mask Callback snap_storage: bitsnap_callback();
      mask TypeOptions snap_dram_dimm: 1 | 2 | 3 | 4
      mask TypeOptions snap_dram_clock: 200 | 250 | 266 | 300 | 333
      mask TypeOptions snap_data_width: 8 | 16 | 32 | 64 | 128
      mask Callback snap_value: bitsnap_callback();
      mask Callback snap_ext_arm: bitsnap_callback();
      mask Callback snap_ext_circ: bitsnap_callback();
      mask Callback snap_provide_outputs: bitsnap_callback();
  spead_pack0 : Subsystem  Tag=casper:spead_pack  AncestorBlock=casper_library_communications/spead_pack  mask(pkt_pack_mask){max_pkt_len_bits=10, header_ids=0x1600, 0x3101, 0x3102, header_ind_ids=0x3300, spead_msw=64, spead_lsw=48, spead_version=4, bytes_per_word=8}
      mask prompts: max_pkt_len_bits "Max pkt length, 2^? 64-bit words"; header_ids "SPEAD direct address IDs (decimal)"; header_ind_ids "SPEAD indirect address IDs (decimal)"; spead_msw "SPEAD Flavour (MSw)"; spead_lsw "SPEAD Flavour (LSw)"; spead_version "SPEAD version"; bytes_per_word "Word size, in bytes"
      mask help:
      | This block generates SPEAD-compliant packets from a datastream.
      |
      | Packets are created with a fixed header followed by a number of 64-bit items.
      |
      | Requires a 64-bit data stream.
      |
      | The data_ready signal is one cycle BEFORE valid data! Does not have to be with a valid signal either.
      mask init:
      | if floor(log2(bytes_per_word)) ~= log2(bytes_per_word)
      |     error('Bytes per word should be a power of two.');
      | end
      | 
      | spead_pack_init(gcb)
  spead_pack1 : Subsystem  Tag=casper:spead_pack  AncestorBlock=casper_library_communications/spead_pack  mask(pkt_pack_mask){max_pkt_len_bits=10, header_ids=0x1600, 0x3101, 0x3102, header_ind_ids=0x3300, spead_msw=64, spead_lsw=48, spead_version=4, bytes_per_word=8}
      mask prompts: max_pkt_len_bits "Max pkt length, 2^? 64-bit words"; header_ids "SPEAD direct address IDs (decimal)"; header_ind_ids "SPEAD indirect address IDs (decimal)"; spead_msw "SPEAD Flavour (MSw)"; spead_lsw "SPEAD Flavour (LSw)"; spead_version "SPEAD version"; bytes_per_word "Word size, in bytes"
      mask help:
      | This block generates SPEAD-compliant packets from a datastream.
      |
      | Packets are created with a fixed header followed by a number of 64-bit items.
      |
      | Requires a 64-bit data stream.
      |
      | The data_ready signal is one cycle BEFORE valid data! Does not have to be with a valid signal either.
      mask init:
      | if floor(log2(bytes_per_word)) ~= log2(bytes_per_word)
      |     error('Bytes per word should be a power of two.');
      | end
      | 
      | spead_pack_init(gcb)
  spead_pack2 : Subsystem  Tag=casper:spead_pack  AncestorBlock=casper_library_communications/spead_pack  mask(pkt_pack_mask){max_pkt_len_bits=10, header_ids=0x1600, 0x3101, 0x3102, header_ind_ids=0x3300, spead_msw=64, spead_lsw=48, spead_version=4, bytes_per_word=8}
      mask prompts: max_pkt_len_bits "Max pkt length, 2^? 64-bit words"; header_ids "SPEAD direct address IDs (decimal)"; header_ind_ids "SPEAD indirect address IDs (decimal)"; spead_msw "SPEAD Flavour (MSw)"; spead_lsw "SPEAD Flavour (LSw)"; spead_version "SPEAD version"; bytes_per_word "Word size, in bytes"
      mask help:
      | This block generates SPEAD-compliant packets from a datastream.
      |
      | Packets are created with a fixed header followed by a number of 64-bit items.
      |
      | Requires a 64-bit data stream.
      |
      | The data_ready signal is one cycle BEFORE valid data! Does not have to be with a valid signal either.
      mask init:
      | if floor(log2(bytes_per_word)) ~= log2(bytes_per_word)
      |     error('Bytes per word should be a power of two.');
      | end
      | 
      | spead_pack_init(gcb)
  spead_pack3 : Subsystem  Tag=casper:spead_pack  AncestorBlock=casper_library_communications/spead_pack  mask(pkt_pack_mask){max_pkt_len_bits=10, header_ids=0x1600, 0x3101, 0x3102, header_ind_ids=0x3300, spead_msw=64, spead_lsw=48, spead_version=4, bytes_per_word=8}
      mask prompts: max_pkt_len_bits "Max pkt length, 2^? 64-bit words"; header_ids "SPEAD direct address IDs (decimal)"; header_ind_ids "SPEAD indirect address IDs (decimal)"; spead_msw "SPEAD Flavour (MSw)"; spead_lsw "SPEAD Flavour (LSw)"; spead_version "SPEAD version"; bytes_per_word "Word size, in bytes"
      mask help:
      | This block generates SPEAD-compliant packets from a datastream.
      |
      | Packets are created with a fixed header followed by a number of 64-bit items.
      |
      | Requires a 64-bit data stream.
      |
      | The data_ready signal is one cycle BEFORE valid data! Does not have to be with a valid signal either.
      mask init:
      | if floor(log2(bytes_per_word)) ~= log2(bytes_per_word)
      |     error('Bytes per word should be a power of two.');
      | end
      | 
      | spead_pack_init(gcb)
  spead_snap0 : Subsystem  Tag=casper:bitsnap  AncestorBlock=casper_library_scopes/bitfield_snapshot  mask(bitsnap){io_names=d64, io_widths=64, io_bps=0, io_types=0, show_format=on, snap_storage=bram, snap_dram_dimm=2, snap_dram_clock=250, snap_nsamples=15, snap_data_width=64, snap_offset=off, snap_circap=off, snap_value=off, snap_ext_arm=off, snap_ext_circ=off, snap_provide_outputs=on, snap_use_dsp48=on, snap_delay=2, extra_names=[c d], extra_widths=[30 2], extra_bps=[0 0], extra_types=[0 0]}
      mask prompts: io_names "Names [msb...lsb]"; io_widths "Bitwidths [msb...lsb]"; io_bps "Binary pts [msb...lsb]"; io_types "Data types [msb...lsb], ufix=0, fix=1, bool=2"; show_format "Print format string?"; snap_storage "Storage medium"; snap_dram_dimm "DRAM dimm"; snap_dram_clock "DRAM clock rate"; snap_nsamples "Number of Samples (2^?)"; snap_data_width "Data width"; snap_offset "Start delay support"; snap_circap "Circular capture support"; snap_value "Extra value capture support"; snap_ext_arm "External arm support"; snap_ext_circ "External circular capture support"; snap_provide_outputs "Provide outputs"; snap_use_dsp48 "Use DSP48s to implement counters"; snap_delay "Pre-snapshot delay"; extra_names "Names [msb...lsb]"; extra_widths "Widths [msb...lsb]"; extra_bps "Binary pts [msb...lsb]"; extra_types "Data types [msb...lsb], ufix=0, fix=1, bool=2"
      mask help:
      | A wrapped snapshot block. Allows specification of inputs to a snapblock word so the toolflow can automatically set up the scope.
      | See documentation for snapshot for explanation of parameters.
      mask init:
      | bitsnap_init(gcb);
      settings: AttributesFormatString=|
      | snap(1):uf64.0 = 64 bits\n64 wide, 32768 deep
      | debugID: 109311942
      mask TypeOptions snap_storage: bram | dram
      mask Callback snap_storage: bitsnap_callback();
      mask TypeOptions snap_dram_dimm: 1 | 2 | 3 | 4
      mask TypeOptions snap_dram_clock: 200 | 250 | 266 | 300 | 333
      mask TypeOptions snap_data_width: 8 | 16 | 32 | 64 | 128
      mask Callback snap_value: bitsnap_callback();
      mask Callback snap_ext_arm: bitsnap_callback();
      mask Callback snap_ext_circ: bitsnap_callback();
      mask Callback snap_provide_outputs: bitsnap_callback();
  speadsnap_control : Subsystem  Tag=xps:sw_reg  AncestorBlock=xps_library/software_register  mask(swreg){io_dir=From Processor, io_delay=0, sample_period=1, names=[speadsnap_arm], bitwidths=1, bin_pts=0, arith_types=2, sim_port=off, show_format=on}
      mask prompts: io_dir "I/O direction"; io_delay "I/O delay"; sample_period "Sample period"; names "Bitfield names [msb...lsb]"; bitwidths "Bitfield widths"; bin_pts "Bitfield binary pts"; arith_types "Bitfield types, ufix=0, fix=1, bool=2"; sim_port "Provide sim input/output?"; show_format "Print format string?"
      mask help: A 32-bit software-accessible register. Can be divided into bitfields of varying widths and types using the fields in the block mask.
      mask init:
      | swreg_init(gcb)
      settings: AttributesFormatString=1input:b = 1 bits
      mask TypeOptions io_dir: To Processor | From Processor
      mask Callback io_dir:
      | mask_enables = get_param(gcb, 'MaskEnables');
      | mask_names = get_param(gcb, 'MaskNames');
      | if strcmp(get_param(gcb, 'io_dir'), 'To Processor'),
      |     mask_enables{ismember(mask_names, 'sample_period')} = 'off';
      | else
      |     mask_enables{ismember(mask_names, 'sample_period')} = 'on';
      | end
      | set_param(gcb, 'MaskEnables', mask_enables);
  speadtime0_offset : Subsystem  Tag=xps:sw_reg  AncestorBlock=xps_library/software_register  mask(swreg){io_dir=From Processor, io_delay=1, sample_period=1, names=speadtime_offset0, bitwidths=32, bin_pts=0, arith_types=0, sim_port=on, show_format=on}
      mask prompts: io_dir "I/O direction"; io_delay "I/O delay"; sample_period "Sample period"; names "Bitfield names [msb...lsb]"; bitwidths "Bitfield widths"; bin_pts "Bitfield binary pts"; arith_types "Bitfield types, ufix=0, fix=1, bool=2"; sim_port "Provide sim input/output?"; show_format "Print format string?"
      mask help: A 32-bit software-accessible register. Can be divided into bitfields of varying widths and types using the fields in the block mask.
      mask init:
      | swreg_init(gcb)
      settings: AttributesFormatString=1input:uf32.0 = 32 bits
      mask TypeOptions io_dir: To Processor | From Processor
      mask Callback io_dir:
      | mask_enables = get_param(gcb, 'MaskEnables');
      | mask_names = get_param(gcb, 'MaskNames');
      | if strcmp(get_param(gcb, 'io_dir'), 'To Processor'),
      |     mask_enables{ismember(mask_names, 'sample_period')} = 'off';
      | else
      |     mask_enables{ismember(mask_names, 'sample_period')} = 'on';
      | end
      | set_param(gcb, 'MaskEnables', mask_enables);
  speadtime1_offset : Subsystem  Tag=xps:sw_reg  AncestorBlock=xps_library/software_register  mask(swreg){io_dir=From Processor, io_delay=1, sample_period=1, names=speadtime_offset1, bitwidths=32, bin_pts=0, arith_types=0, sim_port=on, show_format=on}
      mask prompts: io_dir "I/O direction"; io_delay "I/O delay"; sample_period "Sample period"; names "Bitfield names [msb...lsb]"; bitwidths "Bitfield widths"; bin_pts "Bitfield binary pts"; arith_types "Bitfield types, ufix=0, fix=1, bool=2"; sim_port "Provide sim input/output?"; show_format "Print format string?"
      mask help: A 32-bit software-accessible register. Can be divided into bitfields of varying widths and types using the fields in the block mask.
      mask init:
      | swreg_init(gcb)
      settings: AttributesFormatString=1input:uf32.0 = 32 bits
      mask TypeOptions io_dir: To Processor | From Processor
      mask Callback io_dir:
      | mask_enables = get_param(gcb, 'MaskEnables');
      | mask_names = get_param(gcb, 'MaskNames');
      | if strcmp(get_param(gcb, 'io_dir'), 'To Processor'),
      |     mask_enables{ismember(mask_names, 'sample_period')} = 'off';
      | else
      |     mask_enables{ismember(mask_names, 'sample_period')} = 'on';
      | end
      | set_param(gcb, 'MaskEnables', mask_enables);
  src_sel_cntrl : Subsystem  Tag=xps:sw_reg  AncestorBlock=xps_library/software_register  mask(swreg){io_dir=From Processor, io_delay=1, sample_period=1, names=[src_sel_0 src_sel_1], bitwidths=[2 2], bin_pts=[0 0], arith_types=[0 0], sim_port=on, show_format=on}
      mask prompts: io_dir "I/O direction"; io_delay "I/O delay"; sample_period "Sample period"; names "Bitfield names [msb...lsb]"; bitwidths "Bitfield widths"; bin_pts "Bitfield binary pts"; arith_types "Bitfield types, ufix=0, fix=1, bool=2"; sim_port "Provide sim input/output?"; show_format "Print format string?"
      mask help: A 32-bit software-accessible register. Can be divided into bitfields of varying widths and types using the fields in the block mask.
      mask init:
      | swreg_init(gcb)
      settings: AttributesFormatString=2 inputs:uf2.0,uf2.0 = 4 bits
      mask TypeOptions io_dir: To Processor | From Processor
      mask Callback io_dir:
      | mask_enables = get_param(gcb, 'MaskEnables');
      | mask_names = get_param(gcb, 'MaskNames');
      | if strcmp(get_param(gcb, 'io_dir'), 'To Processor'),
      |     mask_enables{ismember(mask_names, 'sample_period')} = 'off';
      | else
      |     mask_enables{ismember(mask_names, 'sample_period')} = 'on';
      | end
      | set_param(gcb, 'MaskEnables', mask_enables);
  ss_fifo_in : Subsystem  Tag=casper:bitsnap  AncestorBlock=casper_library_scopes/bitfield_snapshot  mask(bitsnap){io_names=[d0 d1 d2 d3 d4 d5 d6 d7 gpio_trig], io_widths=[10 10 10 10 10 10 10 10 1], io_bps=[9 9 9 9 9 9 9 9 0], io_types=[1 1 1 1 1 1 1 1 2], show_format=on, snap_storage=bram, snap_dram_dimm=2, snap_dram_clock=250, snap_nsamples=11, snap_data_width=128, snap_offset=on, snap_circap=off, snap_value=off, snap_ext_arm=off, snap_ext_circ=off, snap_provide_outputs=on, snap_use_dsp48=off, snap_delay=1, extra_names=[c d], extra_widths=[30 2], extra_bps=[0 0], extra_types=[0 0]}
      mask prompts: io_names "Names [msb...lsb]"; io_widths "Bitwidths [msb...lsb]"; io_bps "Binary pts [msb...lsb]"; io_types "Data types [msb...lsb], ufix=0, fix=1, bool=2"; show_format "Print format string?"; snap_storage "Storage medium"; snap_dram_dimm "DRAM dimm"; snap_dram_clock "DRAM clock rate"; snap_nsamples "Number of Samples (2^?)"; snap_data_width "Data width"; snap_offset "Start delay support"; snap_circap "Circular capture support"; snap_value "Extra value capture support"; snap_ext_arm "External arm support"; snap_ext_circ "External circular capture support"; snap_provide_outputs "Provide outputs"; snap_use_dsp48 "Use DSP48s to implement counters"; snap_delay "Pre-snapshot delay"; extra_names "Names [msb...lsb]"; extra_widths "Widths [msb...lsb]"; extra_bps "Binary pts [msb...lsb]"; extra_types "Data types [msb...lsb], ufix=0, fix=1, bool=2"
      mask help:
      | A wrapped snapshot block. Allows specification of inputs to a snapblock word so the toolflow can automatically set up the scope.
      | See documentation for snapshot for explanation of parameters.
      mask init:
      | bitsnap_init(gcb);
      settings: AttributesFormatString=|
      | snap(9):f10.9,f10.9,f10.9,f10.9,f10.9,f10.9,f10.9,f10.9,b = 81 bits\n128 wide, 2048 deep
      | debugID: 19588621
      mask TypeOptions snap_storage: bram | dram
      mask Callback snap_storage: bitsnap_callback();
      mask TypeOptions snap_dram_dimm: 1 | 2 | 3 | 4
      mask TypeOptions snap_dram_clock: 200 | 250 | 266 | 300 | 333
      mask TypeOptions snap_data_width: 8 | 16 | 32 | 64 | 128
      mask Callback snap_value: bitsnap_callback();
      mask Callback snap_ext_arm: bitsnap_callback();
      mask Callback snap_ext_circ: bitsnap_callback();
      mask Callback snap_provide_outputs: bitsnap_callback();
  ss_ip_tx : Subsystem  Tag=casper:bitsnap  AncestorBlock=casper_library_scopes/bitfield_snapshot  mask(bitsnap){io_names=[ip eof dv], io_widths=[32 1 1], io_bps=[0 0 0], io_types=[0 2 2], show_format=on, snap_storage=bram, snap_dram_dimm=2, snap_dram_clock=250, snap_nsamples=13, snap_data_width=64, snap_offset=on, snap_circap=off, snap_value=off, snap_ext_arm=off, snap_ext_circ=off, snap_provide_outputs=on, snap_use_dsp48=off, snap_delay=1, extra_names=[c d], extra_widths=[30 2], extra_bps=[0 0], extra_types=[0 0]}
      mask prompts: io_names "Names [msb...lsb]"; io_widths "Bitwidths [msb...lsb]"; io_bps "Binary pts [msb...lsb]"; io_types "Data types [msb...lsb], ufix=0, fix=1, bool=2"; show_format "Print format string?"; snap_storage "Storage medium"; snap_dram_dimm "DRAM dimm"; snap_dram_clock "DRAM clock rate"; snap_nsamples "Number of Samples (2^?)"; snap_data_width "Data width"; snap_offset "Start delay support"; snap_circap "Circular capture support"; snap_value "Extra value capture support"; snap_ext_arm "External arm support"; snap_ext_circ "External circular capture support"; snap_provide_outputs "Provide outputs"; snap_use_dsp48 "Use DSP48s to implement counters"; snap_delay "Pre-snapshot delay"; extra_names "Names [msb...lsb]"; extra_widths "Widths [msb...lsb]"; extra_bps "Binary pts [msb...lsb]"; extra_types "Data types [msb...lsb], ufix=0, fix=1, bool=2"
      mask help:
      | A wrapped snapshot block. Allows specification of inputs to a snapblock word so the toolflow can automatically set up the scope.
      | See documentation for snapshot for explanation of parameters.
      mask init:
      | bitsnap_init(gcb);
      settings: AttributesFormatString=|
      | snap(3):uf32.0,b,b = 34 bits\n64 wide, 8192 deep
      | debugID: 95752681
      mask TypeOptions snap_storage: bram | dram
      mask Callback snap_storage: bitsnap_callback();
      mask TypeOptions snap_dram_dimm: 1 | 2 | 3 | 4
      mask TypeOptions snap_dram_clock: 200 | 250 | 266 | 300 | 333
      mask TypeOptions snap_data_width: 8 | 16 | 32 | 64 | 128
      mask Callback snap_value: bitsnap_callback();
      mask Callback snap_ext_arm: bitsnap_callback();
      mask Callback snap_ext_circ: bitsnap_callback();
      mask Callback snap_provide_outputs: bitsnap_callback();
  ss_localtime : Subsystem  Tag=casper:bitsnap  AncestorBlock=casper_library_scopes/bitfield_snapshot  mask(bitsnap){io_names=time, io_widths=64, io_bps=0, io_types=0, show_format=on, snap_storage=bram, snap_dram_dimm=2, snap_dram_clock=250, snap_nsamples=11, snap_data_width=64, snap_offset=on, snap_circap=off, snap_value=off, snap_ext_arm=off, snap_ext_circ=off, snap_provide_outputs=on, snap_use_dsp48=off, snap_delay=1, extra_names=[c d], extra_widths=[30 2], extra_bps=[0 0], extra_types=[0 0]}
      mask prompts: io_names "Names [msb...lsb]"; io_widths "Bitwidths [msb...lsb]"; io_bps "Binary pts [msb...lsb]"; io_types "Data types [msb...lsb], ufix=0, fix=1, bool=2"; show_format "Print format string?"; snap_storage "Storage medium"; snap_dram_dimm "DRAM dimm"; snap_dram_clock "DRAM clock rate"; snap_nsamples "Number of Samples (2^?)"; snap_data_width "Data width"; snap_offset "Start delay support"; snap_circap "Circular capture support"; snap_value "Extra value capture support"; snap_ext_arm "External arm support"; snap_ext_circ "External circular capture support"; snap_provide_outputs "Provide outputs"; snap_use_dsp48 "Use DSP48s to implement counters"; snap_delay "Pre-snapshot delay"; extra_names "Names [msb...lsb]"; extra_widths "Widths [msb...lsb]"; extra_bps "Binary pts [msb...lsb]"; extra_types "Data types [msb...lsb], ufix=0, fix=1, bool=2"
      mask help:
      | A wrapped snapshot block. Allows specification of inputs to a snapblock word so the toolflow can automatically set up the scope.
      | See documentation for snapshot for explanation of parameters.
      mask init:
      | bitsnap_init(gcb);
      settings: AttributesFormatString=|
      | snap(1):uf64.0 = 64 bits\n64 wide, 2048 deep
      | debugID: 69418317
      mask TypeOptions snap_storage: bram | dram
      mask Callback snap_storage: bitsnap_callback();
      mask TypeOptions snap_dram_dimm: 1 | 2 | 3 | 4
      mask TypeOptions snap_dram_clock: 200 | 250 | 266 | 300 | 333
      mask TypeOptions snap_data_width: 8 | 16 | 32 | 64 | 128
      mask Callback snap_value: bitsnap_callback();
      mask Callback snap_ext_arm: bitsnap_callback();
      mask Callback snap_ext_circ: bitsnap_callback();
      mask Callback snap_provide_outputs: bitsnap_callback();
  ss_trig_time_lsw : Subsystem  Tag=xps:sw_reg  AncestorBlock=xps_library/software_register  mask(swreg){io_dir=From Processor, io_delay=1, sample_period=1, names=reg, bitwidths=32, bin_pts=0, arith_types=0, sim_port=on, show_format=on}
      mask prompts: io_dir "I/O direction"; io_delay "I/O delay"; sample_period "Sample period"; names "Bitfield names [msb...lsb]"; bitwidths "Bitfield widths"; bin_pts "Bitfield binary pts"; arith_types "Bitfield types, ufix=0, fix=1, bool=2"; sim_port "Provide sim input/output?"; show_format "Print format string?"
      mask help: A 32-bit software-accessible register. Can be divided into bitfields of varying widths and types using the fields in the block mask.
      mask init:
      | swreg_init(gcb)
      settings: AttributesFormatString=1input:uf32.0 = 32 bits
      mask TypeOptions io_dir: To Processor | From Processor
      mask Callback io_dir:
      | mask_enables = get_param(gcb, 'MaskEnables');
      | mask_names = get_param(gcb, 'MaskNames');
      | if strcmp(get_param(gcb, 'io_dir'), 'To Processor'),
      |     mask_enables{ismember(mask_names, 'sample_period')} = 'off';
      | else
      |     mask_enables{ismember(mask_names, 'sample_period')} = 'on';
      | end
      | set_param(gcb, 'MaskEnables', mask_enables);
  ss_trig_time_msw : Subsystem  Tag=xps:sw_reg  AncestorBlock=xps_library/software_register  mask(swreg){io_dir=From Processor, io_delay=1, sample_period=1, names=reg, bitwidths=32, bin_pts=0, arith_types=0, sim_port=on, show_format=on}
      mask prompts: io_dir "I/O direction"; io_delay "I/O delay"; sample_period "Sample period"; names "Bitfield names [msb...lsb]"; bitwidths "Bitfield widths"; bin_pts "Bitfield binary pts"; arith_types "Bitfield types, ufix=0, fix=1, bool=2"; sim_port "Provide sim input/output?"; show_format "Print format string?"
      mask help: A 32-bit software-accessible register. Can be divided into bitfields of varying widths and types using the fields in the block mask.
      mask init:
      | swreg_init(gcb)
      settings: AttributesFormatString=1input:uf32.0 = 32 bits
      mask TypeOptions io_dir: To Processor | From Processor
      mask Callback io_dir:
      | mask_enables = get_param(gcb, 'MaskEnables');
      | mask_names = get_param(gcb, 'MaskNames');
      | if strcmp(get_param(gcb, 'io_dir'), 'To Processor'),
      |     mask_enables{ismember(mask_names, 'sample_period')} = 'off';
      | else
      |     mask_enables{ismember(mask_names, 'sample_period')} = 'on';
      | end
      | set_param(gcb, 'MaskEnables', mask_enables);
  start_flag_lsw : Subsystem  Tag=xps:sw_reg  AncestorBlock=xps_library/software_register  mask(swreg){io_dir=From Processor, io_delay=1, sample_period=1, names=reg, bitwidths=32, bin_pts=0, arith_types=0, sim_port=on, show_format=on}
      mask prompts: io_dir "I/O direction"; io_delay "I/O delay"; sample_period "Sample period"; names "Bitfield names [msb...lsb]"; bitwidths "Bitfield widths"; bin_pts "Bitfield binary pts"; arith_types "Bitfield types, ufix=0, fix=1, bool=2"; sim_port "Provide sim input/output?"; show_format "Print format string?"
      mask help: A 32-bit software-accessible register. Can be divided into bitfields of varying widths and types using the fields in the block mask.
      mask init:
      | swreg_init(gcb)
      settings: AttributesFormatString=1input:uf32.0 = 32 bits
      mask TypeOptions io_dir: To Processor | From Processor
      mask Callback io_dir:
      | mask_enables = get_param(gcb, 'MaskEnables');
      | mask_names = get_param(gcb, 'MaskNames');
      | if strcmp(get_param(gcb, 'io_dir'), 'To Processor'),
      |     mask_enables{ismember(mask_names, 'sample_period')} = 'off';
      | else
      |     mask_enables{ismember(mask_names, 'sample_period')} = 'on';
      | end
      | set_param(gcb, 'MaskEnables', mask_enables);
  start_flag_msw : Subsystem  Tag=xps:sw_reg  AncestorBlock=xps_library/software_register  mask(swreg){io_dir=From Processor, io_delay=1, sample_period=1, names=reg, bitwidths=32, bin_pts=0, arith_types=0, sim_port=on, show_format=on}
      mask prompts: io_dir "I/O direction"; io_delay "I/O delay"; sample_period "Sample period"; names "Bitfield names [msb...lsb]"; bitwidths "Bitfield widths"; bin_pts "Bitfield binary pts"; arith_types "Bitfield types, ufix=0, fix=1, bool=2"; sim_port "Provide sim input/output?"; show_format "Print format string?"
      mask help: A 32-bit software-accessible register. Can be divided into bitfields of varying widths and types using the fields in the block mask.
      mask init:
      | swreg_init(gcb)
      settings: AttributesFormatString=1input:uf32.0 = 32 bits
      mask TypeOptions io_dir: To Processor | From Processor
      mask Callback io_dir:
      | mask_enables = get_param(gcb, 'MaskEnables');
      | mask_names = get_param(gcb, 'MaskNames');
      | if strcmp(get_param(gcb, 'io_dir'), 'To Processor'),
      |     mask_enables{ismember(mask_names, 'sample_period')} = 'off';
      | else
      |     mask_enables{ismember(mask_names, 'sample_period')} = 'on';
      | end
      | set_param(gcb, 'MaskEnables', mask_enables);
  start_load_time_lsw : Subsystem  Tag=xps:sw_reg  AncestorBlock=xps_library/software_register  mask(swreg){io_dir=From Processor, io_delay=1, sample_period=1, names=reg, bitwidths=32, bin_pts=0, arith_types=0, sim_port=on, show_format=on}
      mask prompts: io_dir "I/O direction"; io_delay "I/O delay"; sample_period "Sample period"; names "Bitfield names [msb...lsb]"; bitwidths "Bitfield widths"; bin_pts "Bitfield binary pts"; arith_types "Bitfield types, ufix=0, fix=1, bool=2"; sim_port "Provide sim input/output?"; show_format "Print format string?"
      mask help: A 32-bit software-accessible register. Can be divided into bitfields of varying widths and types using the fields in the block mask.
      mask init:
      | swreg_init(gcb)
      settings: AttributesFormatString=1input:uf32.0 = 32 bits
      mask TypeOptions io_dir: To Processor | From Processor
      mask Callback io_dir:
      | mask_enables = get_param(gcb, 'MaskEnables');
      | mask_names = get_param(gcb, 'MaskNames');
      | if strcmp(get_param(gcb, 'io_dir'), 'To Processor'),
      |     mask_enables{ismember(mask_names, 'sample_period')} = 'off';
      | else
      |     mask_enables{ismember(mask_names, 'sample_period')} = 'on';
      | end
      | set_param(gcb, 'MaskEnables', mask_enables);
  start_load_time_msw : Subsystem  Tag=xps:sw_reg  AncestorBlock=xps_library/software_register  mask(swreg){io_dir=From Processor, io_delay=1, sample_period=1, names=reg, bitwidths=32, bin_pts=0, arith_types=0, sim_port=on, show_format=on}
      mask prompts: io_dir "I/O direction"; io_delay "I/O delay"; sample_period "Sample period"; names "Bitfield names [msb...lsb]"; bitwidths "Bitfield widths"; bin_pts "Bitfield binary pts"; arith_types "Bitfield types, ufix=0, fix=1, bool=2"; sim_port "Provide sim input/output?"; show_format "Print format string?"
      mask help: A 32-bit software-accessible register. Can be divided into bitfields of varying widths and types using the fields in the block mask.
      mask init:
      | swreg_init(gcb)
      settings: AttributesFormatString=1input:uf32.0 = 32 bits
      mask TypeOptions io_dir: To Processor | From Processor
      mask Callback io_dir:
      | mask_enables = get_param(gcb, 'MaskEnables');
      | mask_names = get_param(gcb, 'MaskNames');
      | if strcmp(get_param(gcb, 'io_dir'), 'To Processor'),
      |     mask_enables{ismember(mask_names, 'sample_period')} = 'off';
      | else
      |     mask_enables{ismember(mask_names, 'sample_period')} = 'on';
      | end
      | set_param(gcb, 'MaskEnables', mask_enables);
  start_stop_cntrl : Subsystem
  start_stop_ctr : Subsystem  Tag=xps:sw_reg  AncestorBlock=xps_library/software_register  mask(swreg){io_dir=To Processor, io_delay=1, sample_period=1, names=reg, bitwidths=32, bin_pts=0, arith_types=0, sim_port=off, show_format=on}
      mask prompts: io_dir "I/O direction"; io_delay "I/O delay"; sample_period "Sample period"; names "Bitfield names [msb...lsb]"; bitwidths "Bitfield widths"; bin_pts "Bitfield binary pts"; arith_types "Bitfield types, ufix=0, fix=1, bool=2"; sim_port "Provide sim input/output?"; show_format "Print format string?"
      mask help: A 32-bit software-accessible register. Can be divided into bitfields of varying widths and types using the fields in the block mask.
      mask init:
      | swreg_init(gcb)
      settings: AttributesFormatString=1output:uf32.0 = 32 bits
      mask TypeOptions io_dir: To Processor | From Processor
      mask Callback io_dir:
      | mask_enables = get_param(gcb, 'MaskEnables');
      | mask_names = get_param(gcb, 'MaskNames');
      | if strcmp(get_param(gcb, 'io_dir'), 'To Processor'),
      |     mask_enables{ismember(mask_names, 'sample_period')} = 'off';
      | else
      |     mask_enables{ismember(mask_names, 'sample_period')} = 'on';
      | end
      | set_param(gcb, 'MaskEnables', mask_enables);
  start_time_lsw : Subsystem  Tag=xps:sw_reg  AncestorBlock=xps_library/software_register  mask(swreg){io_dir=From Processor, io_delay=1, sample_period=1, names=reg, bitwidths=32, bin_pts=0, arith_types=0, sim_port=on, show_format=on}
      mask prompts: io_dir "I/O direction"; io_delay "I/O delay"; sample_period "Sample period"; names "Bitfield names [msb...lsb]"; bitwidths "Bitfield widths"; bin_pts "Bitfield binary pts"; arith_types "Bitfield types, ufix=0, fix=1, bool=2"; sim_port "Provide sim input/output?"; show_format "Print format string?"
      mask help: A 32-bit software-accessible register. Can be divided into bitfields of varying widths and types using the fields in the block mask.
      mask init:
      | swreg_init(gcb)
      settings: AttributesFormatString=1input:uf32.0 = 32 bits
      mask TypeOptions io_dir: To Processor | From Processor
      mask Callback io_dir:
      | mask_enables = get_param(gcb, 'MaskEnables');
      | mask_names = get_param(gcb, 'MaskNames');
      | if strcmp(get_param(gcb, 'io_dir'), 'To Processor'),
      |     mask_enables{ismember(mask_names, 'sample_period')} = 'off';
      | else
      |     mask_enables{ismember(mask_names, 'sample_period')} = 'on';
      | end
      | set_param(gcb, 'MaskEnables', mask_enables);
  start_time_msw : Subsystem  Tag=xps:sw_reg  AncestorBlock=xps_library/software_register  mask(swreg){io_dir=From Processor, io_delay=1, sample_period=1, names=reg, bitwidths=32, bin_pts=0, arith_types=0, sim_port=on, show_format=on}
      mask prompts: io_dir "I/O direction"; io_delay "I/O delay"; sample_period "Sample period"; names "Bitfield names [msb...lsb]"; bitwidths "Bitfield widths"; bin_pts "Bitfield binary pts"; arith_types "Bitfield types, ufix=0, fix=1, bool=2"; sim_port "Provide sim input/output?"; show_format "Print format string?"
      mask help: A 32-bit software-accessible register. Can be divided into bitfields of varying widths and types using the fields in the block mask.
      mask init:
      | swreg_init(gcb)
      settings: AttributesFormatString=1input:uf32.0 = 32 bits
      mask TypeOptions io_dir: To Processor | From Processor
      mask Callback io_dir:
      | mask_enables = get_param(gcb, 'MaskEnables');
      | mask_names = get_param(gcb, 'MaskNames');
      | if strcmp(get_param(gcb, 'io_dir'), 'To Processor'),
      |     mask_enables{ismember(mask_names, 'sample_period')} = 'off';
      | else
      |     mask_enables{ismember(mask_names, 'sample_period')} = 'on';
      | end
      | set_param(gcb, 'MaskEnables', mask_enables);
  status0 : Subsystem  Tag=xps:sw_reg  AncestorBlock=xps_library/software_register  mask(swreg){io_dir=To Processor, io_delay=0, sample_period=1, names=[led_up led_rx led_tx tx_afull tx_overflow rx_overrun], bitwidths=1, bin_pts=0, arith_types=2, sim_port=off, show_format=on}
      mask prompts: io_dir "I/O direction"; io_delay "I/O delay"; sample_period "Sample period"; names "Bitfield names [msb...lsb]"; bitwidths "Bitfield widths"; bin_pts "Bitfield binary pts"; arith_types "Bitfield types, ufix=0, fix=1, bool=2"; sim_port "Provide sim input/output?"; show_format "Print format string?"
      mask help: A 32-bit software-accessible register. Can be divided into bitfields of varying widths and types using the fields in the block mask.
      mask init:
      | swreg_init(gcb)
      settings: AttributesFormatString=6 outputs:b,b,b,b,b,b = 6 bits
      mask TypeOptions io_dir: To Processor | From Processor
      mask Callback io_dir:
      | mask_enables = get_param(gcb, 'MaskEnables');
      | mask_names = get_param(gcb, 'MaskNames');
      | if strcmp(get_param(gcb, 'io_dir'), 'To Processor'),
      |     mask_enables{ismember(mask_names, 'sample_period')} = 'off';
      | else
      |     mask_enables{ismember(mask_names, 'sample_period')} = 'on';
      | end
      | set_param(gcb, 'MaskEnables', mask_enables);
  stop_load_time_lsw : Subsystem  Tag=xps:sw_reg  AncestorBlock=xps_library/software_register  mask(swreg){io_dir=From Processor, io_delay=1, sample_period=1, names=reg, bitwidths=32, bin_pts=0, arith_types=0, sim_port=on, show_format=on}
      mask prompts: io_dir "I/O direction"; io_delay "I/O delay"; sample_period "Sample period"; names "Bitfield names [msb...lsb]"; bitwidths "Bitfield widths"; bin_pts "Bitfield binary pts"; arith_types "Bitfield types, ufix=0, fix=1, bool=2"; sim_port "Provide sim input/output?"; show_format "Print format string?"
      mask help: A 32-bit software-accessible register. Can be divided into bitfields of varying widths and types using the fields in the block mask.
      mask init:
      | swreg_init(gcb)
      settings: AttributesFormatString=1input:uf32.0 = 32 bits
      mask TypeOptions io_dir: To Processor | From Processor
      mask Callback io_dir:
      | mask_enables = get_param(gcb, 'MaskEnables');
      | mask_names = get_param(gcb, 'MaskNames');
      | if strcmp(get_param(gcb, 'io_dir'), 'To Processor'),
      |     mask_enables{ismember(mask_names, 'sample_period')} = 'off';
      | else
      |     mask_enables{ismember(mask_names, 'sample_period')} = 'on';
      | end
      | set_param(gcb, 'MaskEnables', mask_enables);
  stop_load_time_msw : Subsystem  Tag=xps:sw_reg  AncestorBlock=xps_library/software_register  mask(swreg){io_dir=From Processor, io_delay=1, sample_period=1, names=reg, bitwidths=32, bin_pts=0, arith_types=0, sim_port=on, show_format=on}
      mask prompts: io_dir "I/O direction"; io_delay "I/O delay"; sample_period "Sample period"; names "Bitfield names [msb...lsb]"; bitwidths "Bitfield widths"; bin_pts "Bitfield binary pts"; arith_types "Bitfield types, ufix=0, fix=1, bool=2"; sim_port "Provide sim input/output?"; show_format "Print format string?"
      mask help: A 32-bit software-accessible register. Can be divided into bitfields of varying widths and types using the fields in the block mask.
      mask init:
      | swreg_init(gcb)
      settings: AttributesFormatString=1input:uf32.0 = 32 bits
      mask TypeOptions io_dir: To Processor | From Processor
      mask Callback io_dir:
      | mask_enables = get_param(gcb, 'MaskEnables');
      | mask_names = get_param(gcb, 'MaskNames');
      | if strcmp(get_param(gcb, 'io_dir'), 'To Processor'),
      |     mask_enables{ismember(mask_names, 'sample_period')} = 'off';
      | else
      |     mask_enables{ismember(mask_names, 'sample_period')} = 'on';
      | end
      | set_param(gcb, 'MaskEnables', mask_enables);
  tick_offset_lsw : Subsystem  Tag=xps:sw_reg  AncestorBlock=xps_library/software_register  mask(swreg){io_dir=From Processor, io_delay=1, sample_period=1, names=reg, bitwidths=32, bin_pts=0, arith_types=0, sim_port=on, show_format=on}
      mask prompts: io_dir "I/O direction"; io_delay "I/O delay"; sample_period "Sample period"; names "Bitfield names [msb...lsb]"; bitwidths "Bitfield widths"; bin_pts "Bitfield binary pts"; arith_types "Bitfield types, ufix=0, fix=1, bool=2"; sim_port "Provide sim input/output?"; show_format "Print format string?"
      mask help: A 32-bit software-accessible register. Can be divided into bitfields of varying widths and types using the fields in the block mask.
      mask init:
      | swreg_init(gcb)
      settings: AttributesFormatString=1input:uf32.0 = 32 bits
      mask TypeOptions io_dir: To Processor | From Processor
      mask Callback io_dir:
      | mask_enables = get_param(gcb, 'MaskEnables');
      | mask_names = get_param(gcb, 'MaskNames');
      | if strcmp(get_param(gcb, 'io_dir'), 'To Processor'),
      |     mask_enables{ismember(mask_names, 'sample_period')} = 'off';
      | else
      |     mask_enables{ismember(mask_names, 'sample_period')} = 'on';
      | end
      | set_param(gcb, 'MaskEnables', mask_enables);
  tick_offset_msw : Subsystem  Tag=xps:sw_reg  AncestorBlock=xps_library/software_register  mask(swreg){io_dir=From Processor, io_delay=1, sample_period=1, names=reg, bitwidths=32, bin_pts=0, arith_types=0, sim_port=on, show_format=on}
      mask prompts: io_dir "I/O direction"; io_delay "I/O delay"; sample_period "Sample period"; names "Bitfield names [msb...lsb]"; bitwidths "Bitfield widths"; bin_pts "Bitfield binary pts"; arith_types "Bitfield types, ufix=0, fix=1, bool=2"; sim_port "Provide sim input/output?"; show_format "Print format string?"
      mask help: A 32-bit software-accessible register. Can be divided into bitfields of varying widths and types using the fields in the block mask.
      mask init:
      | swreg_init(gcb)
      settings: AttributesFormatString=1input:uf32.0 = 32 bits
      mask TypeOptions io_dir: To Processor | From Processor
      mask Callback io_dir:
      | mask_enables = get_param(gcb, 'MaskEnables');
      | mask_names = get_param(gcb, 'MaskNames');
      | if strcmp(get_param(gcb, 'io_dir'), 'To Processor'),
      |     mask_enables{ismember(mask_names, 'sample_period')} = 'off';
      | else
      |     mask_enables{ismember(mask_names, 'sample_period')} = 'on';
      | end
      | set_param(gcb, 'MaskEnables', mask_enables);
  ticks_since_mrst : Subsystem
  tvg_spead_time_with_pkt_ctr : Subsystem  mask{packetlen_bits=9}
      mask prompts: packetlen_bits "Packet length, num 80-bit words (2^?):"
  tx_gate_ctrs : Subsystem  Tag=xps:sw_reg  AncestorBlock=xps_library/software_register  mask(swreg){io_dir=To Processor, io_delay=1, sample_period=1, names=sp0 sp1 sp2 sp3, bitwidths=8, bin_pts=0, arith_types=0, sim_port=off, show_format=on}
      mask prompts: io_dir "I/O direction"; io_delay "I/O delay"; sample_period "Sample period"; names "Bitfield names [msb...lsb]"; bitwidths "Bitfield widths"; bin_pts "Bitfield binary pts"; arith_types "Bitfield types, ufix=0, fix=1, bool=2"; sim_port "Provide sim input/output?"; show_format "Print format string?"
      mask help: A 32-bit software-accessible register. Can be divided into bitfields of varying widths and types using the fields in the block mask.
      mask init:
      | swreg_init(gcb)
      settings: AttributesFormatString=4 outputs:uf8.0,uf8.0,uf8.0,uf8.0 = 32 bits
      mask TypeOptions io_dir: To Processor | From Processor
      mask Callback io_dir:
      | mask_enables = get_param(gcb, 'MaskEnables');
      | mask_names = get_param(gcb, 'MaskNames');
      | if strcmp(get_param(gcb, 'io_dir'), 'To Processor'),
      |     mask_enables{ismember(mask_names, 'sample_period')} = 'off';
      | else
      |     mask_enables{ismember(mask_names, 'sample_period')} = 'on';
      | end
      | set_param(gcb, 'MaskEnables', mask_enables);
  wng0 : Subsystem  mask{seed1=hex2dec('12345678'), seed2=hex2dec('87654321'), seed3=hex2dec('45612378'), seed4=hex2dec('85274163')}
      mask prompts: seed1 "Seed 1"; seed2 "Seed 2"; seed3 "Seed 3"; seed4 "Seed 4"
  wng1 : Subsystem  mask{seed1=hex2dec('65498732'), seed2=hex2dec('32198754'), seed3=hex2dec('56123784'), seed4=hex2dec('74563218')}
      mask prompts: seed1 "Seed 1"; seed2 "Seed 2"; seed3 "Seed 3"; seed4 "Seed 4"
  wng_corr : Subsystem  mask{seed1=hex2dec('75386429'), seed2=hex2dec('95123754'), seed3=hex2dec('98321495'), seed4=hex2dec('96478521')}
      mask prompts: seed1 "Seed 1"; seed2 "Seed 2"; seed3 "Seed 3"; seed4 "Seed 4"
  wng_rst : Subsystem
  wr_addr{0..3} (4 alike) : xbsIndex_r4/Counter  cnt_type=Free Running  cnt_to=Inf  operation=Up  start_count=0  cnt_by_val=1  arith_type=Unsigned  n_bits=10  bin_pt=0  load_pin=off  rst=on  en=on  explicit_period=on  period=1  use_behavioral_HDL=off  implementation=Fabric  dbl_ovrd=off  block_type=counter
  tag scope: arb_en0=global, arb_rst0=global, cnt_rst=global, dram_addr_offset0=global, dram_rd_repeat0=global, dram_rd_repeat_delay0=global, dram_rd_trig0=global, dram_read_length0=global, dram_tvg0=global, dram_tvg_length0=global, local_time=global, spead_data0=global, spead_data1=global, spead_data2=global, spead_data3=global, spead_eof0=global, spead_eof1=global, spead_eof2=global, spead_eof3=global, spead_valid0=global, spead_valid1=global, spead_valid2=global, spead_valid3=global, tvg_sel0=global
  wires:
  [tvg_select0] -> Delay102/1
  Mux/1 -> Assert/1  "d80_0"
  fifo0/1(fifo_data80) -> pipeline96/1(d)  "data00"
  fifo0/2(fifo_dv) -> pipeline97/1(d)  "dv00"
  fifo0/3(word_start) -> pipeline98/1(d)  "ws00"
  fifo0/4(pkt_start) -> pipeline99/1(d)  "ps00"
  gbe_porttx/1(in_reg) -> pipeline15/1(d)
  Constant9/1 -> gbe_porttx/1(sim_1)
  Constant15/1 -> digitiser_id/1(sim_1)
  Constant17/1 -> receptor_id/1(sim_1)
  fifo0/5(fifo_full) -> Terminator16/1  "full00"
  fifo0/6(fifo_empty) -> Terminator23/1  "empty00"
  fifo1/1(fifo_data80) -> pipeline100/1(d)  "data01"
  fifo1/2(fifo_dv) -> pipeline101/1(d)  "dv01"
  fifo1/3(word_start) -> pipeline102/1(d)  "ws01"
  fifo1/4(pkt_start) -> pipeline103/1(d)  "ps01"
  pack_80_64_1/3(data64) -> pipeline117/1(d)  "d64_00"
  pack_80_64_1/2(valid64) -> Gateway Out84/1, pipeline116/1(d)  "v64_01"
  pack_80_64_1/1(ready64) -> pipeline115/1(d)  "r64_01"
  fifo1/5(fifo_full) -> Terminator18/1
  fifo1/6(fifo_empty) -> Terminator20/1
  Constant16/1 -> digitiser_id/2(sim_2)
  receptor_id/1(in_receptor_id) -> bus_create/3(in3)
  Constant6/1 -> receptor_id/2(sim_2)
  Constant19/1 -> receptor_id/3(sim_3)
  [hdr_0x3101] -> bus_create9/1(in1)
  [pol0_id] -> bus_create9/2(in2)
  [hdr_0x3101] -> bus_create1/1(in1)
  [pol0_id] -> bus_create1/2(in2)
  [speadtime0] -> spead_pack0/8(hdr5_0x1600_DIR), spead_pack0/4(hdr_heap_id)  "timein0"
  bus_create9/1(bus_out) -> spead_pack0/9(hdr6_0x3101_DIR)
  [status0] -> spead_pack0/10(hdr7_0x3102_DIR)
  bus_create1/1(bus_out) -> spead_pack1/9(hdr6_0x3101_DIR)
  [status1] -> spead_pack1/10(hdr7_0x3102_DIR)
  [tvg_ltime] -> Gateway Out93/1, fifo_select/1(localtime)
  fifo_select/1(select) -> Delay3/1  "fifo_select"
  Delay3/1 -> [fifoselect], Gateway Out91/1, Inverter/1, fifo0/2(fifo_we_en)  "fifoselect"
  [speadtime1] -> spead_pack1/4(hdr_heap_id), spead_pack1/8(hdr5_0x1600_DIR)  "timein1"
  pack_80_64_00/1(ready64) -> pipeline112/1(d)  "r64_00"
  pack_80_64_00/2(valid64) -> pipeline113/1(d)  "v64_00"
  [spead_heapsize] -> spead_pack0/5(hdr_heap_size)
  [spead_heapoffset] -> spead_pack0/6(hdr_heap_offset)
  [spead_pktlen] -> spead_pack0/7(hdr_pkt_len_words)
  [spead_heapsize] -> spead_pack1/5(hdr_heap_size)
  [spead_heapoffset] -> spead_pack1/6(hdr_heap_offset)
  [spead_pktlen] -> spead_pack1/7(hdr_pkt_len_words)
  [masked_time] -> Delay128/1
  Assert/1 -> bus_expand5/1(bus_in), fifo1/1(data80), fifo0/1(data80)
  tvg_spead_time_with_pkt_ctr/1(local_time) -> Delay131/1
  tvg_spead_time_with_pkt_ctr/3(tvg_data_pol0) -> Delay133/1
  tvg_spead_time_with_pkt_ctr/4(tvg_data_pol1) -> Delay134/1
  tvg_spead_time_with_pkt_ctr/2(spead_time) -> Delay132/1
  spead_pack1/4(data_overflow) -> Terminator15/1
  [adc_data_offset] -> spead_pack0/11(hdr8_0x3300)
  [adc_data_offset] -> spead_pack1/11(hdr8_0x3300)
  spead_pack0/4(data_overflow) -> Terminator12/1
  spead_pack0/3(eof) -> pipeline56/1(d)
  spead_pack0/1(data_out) -> pipeline54/1(d)  "packd"
  spead_pack0/2(valid_out) -> pipeline55/1(d)  "packv"
  spead_pack1/1(data_out) -> pipeline57/1(d)
  spead_pack1/2(valid_out) -> pipeline58/1(d)
  spead_pack1/3(eof) -> pipeline59/1(d)
  [fifoselect] -> edge_detect5/1(in), Inverter2/1
  Register5/1 -> [speadtime0]  "speadtime0"
  Inverter2/1 -> edge_detect6/1(in)
  edge_detect5/1(out) -> Register5/2
  edge_detect6/1(out) -> Register6/2
  Register6/1 -> [speadtime1]  "speadtime1"
  ticks_since_mrst/1(time64) -> Gateway Out97/1, [local_time]  "localtime"
  edge_detect2/1(out) -> [mrst]  "mrst"
  edge_detect1/1(out) -> [msync]  "msync"
  edge_detect4/1(out) -> [clr_status]  "clr_status"
  [local_time] -> slice1/1, slice2/1
  [tick_offset] -> Gateway Out100/1, ticks_since_mrst/3(offset)
  edge_detect10/1(out) -> [load_tick_offset]  "mrst"
  digitiser_id/1(in_digitiser_serial) -> bus_create/1(in1)
  digitiser_id/2(in_digitiser_type) -> bus_create/2(in2)
  Constant43/1 -> flag_setup/3(sim_3)
  Constant42/1 -> flag_setup/2(sim_2)
  Constant39/1 -> flag_setup/1(sim_1)
  Counter Free-Running3/1 -> Relational Operator4/2
  Constant48/1 -> Relational Operator4/1
  Relational Operator4/1 -> flag_setup/4(sim_4)
  Constant52/1 -> start_flag_msw/1(sim_1)
  Constant53/1 -> start_flag_lsw/1(sim_1)
  Constant51/1 -> end_flag_msw/1(sim_1)
  Constant50/1 -> end_flag_lsw/1(sim_1)
  Concat4/1 -> Delay49/1  "starttime"
  Concat5/1 -> Delay50/1  "stoptime"
  [flag_start_time] -> Delay46/1
  [local_time] -> Delay45/1, Delay47/1
  [flag_end_time] -> Delay48/1, Delay51/1
  Relational/1 -> Logical2/2  "start_okay"
  [flag_armed] -> Delay44/1
  Relational1/1 -> Logical4/2  "end_okay"
  Logical2/1 -> Delay23/1  "start_okay"
  Logical4/1 -> Logical3/1  "end_okay"
  edge_detect9/1(out) -> [load_flag_time]  "loadtimes"
  Constant4/1 -> Register1/1
  edge_detect8/1(out) -> [reset_flag_time]  "rst"
  [reset_flag_time] -> Register1/2
  [load_flag_time] -> Register1/3
  Register1/1 -> [flag_armed]  "armed"
  Relational Operator3/1 -> flag_setup/5(sim_5)
  Relational2/1 -> Delay22/1  "zero_stop"
  Constant2/1 -> Relational2/2
  Logical3/1 -> Logical1/2  "eokay"
  Counter Free-Running2/1 -> Relational Operator3/2
  Constant5/1 -> Relational Operator3/1
  Logical5/1 -> sample_masking/2(den_in)
  Constant49/1 -> start_time_msw/1(sim_1)
  Constant54/1 -> start_time_lsw/1(sim_1)
  Constant3/1 -> end_time_msw/1(sim_1)
  Constant11/1 -> end_time_lsw/1(sim_1)
  Relational3/1 -> Logical6/2  "start_okay"
  Relational4/1 -> Logical8/2  "end_okay"
  [start_time] -> Delay39/1
  Relational6/1 -> Delay15/1  "first_sample"
  [end_time] -> Delay41/1
  Relational7/1 -> Delay16/1  "last_sample"
  [sample_end] -> sample_masking/6(sample_end)
  [sample_start] -> sample_masking/5(sample_start)
  sample_masking/2(den_out) -> Delay126/1  "enable"
  sample_masking/3(data_mask) -> Delay127/1  "mask"
  edge_detect11/1(out) -> [reset_en_time]  "reset_en_time"
  Relational Operator5/1 -> control_output/2(sim_2)
  Counter Free-Running4/1 -> Relational Operator5/2, Relational Operator6/2
  Constant38/1 -> Relational Operator5/1
  edge_detect12/1(out) -> [load_en_time]  "load_en_time"
  Concat/1 -> Delay42/1
  Concat1/1 -> Delay43/1
  Constant22/1 -> Register2/1
  [reset_en_time] -> Register2/2
  [load_en_time] -> Register2/3
  Register2/1 -> [en_armed]  "armed"
  Logical6/1 -> Delay17/1  "start_okay"
  Logical8/1 -> Logical7/1  "end_okay"
  Logical7/1 -> Logical5/2
  Constant34/1 -> Delay37/1
  Relational5/1 -> Delay14/1
  Constant29/1 -> control_output/3(sim_3)
  Constant47/1 -> control_output/4(sim_4)
  Constant31/1 -> Relational Operator6/1
  Relational Operator6/1 -> control_output/1(sim_1)
  [data_enable] -> Delay129/1
  [sample_mask] -> Delay130/1
  Constant46/1 -> tick_offset_msw/1(sim_1)
  Constant7/1 -> tick_offset_lsw/1(sim_1)
  Concat2/1 -> Register3/1
  [load_tick_offset] -> Register3/2
  Register3/1 -> [tick_offset]
  fifo2/1(fifo_data80) -> pipeline104/1(d)  "data00"
  fifo2/2(fifo_dv) -> pipeline105/1(d)  "dv00"
  fifo2/3(word_start) -> pipeline106/1(d)  "ws00"
  fifo2/4(pkt_start) -> pipeline107/1(d)  "ps00"
  fifo2/5(fifo_full) -> Terminator3/1  "full00"
  fifo2/6(fifo_empty) -> Terminator6/1  "empty00"
  fifo3/1(fifo_data80) -> pipeline108/1(d)  "data01"
  fifo3/2(fifo_dv) -> pipeline109/1(d)  "dv01"
  fifo3/3(word_start) -> pipeline110/1(d)  "ws01"
  fifo3/4(pkt_start) -> pipeline111/1(d)  "ps01"
  pack_80_64_3/3(data64) -> pipeline123/1(d)  "d64_00"
  pack_80_64_3/2(valid64) -> Gateway Out83/1, pipeline122/1(d)  "v64_01"
  pack_80_64_3/1(ready64) -> pipeline121/1(d)  "r64_01"
  fifo3/5(fifo_full) -> Terminator4/1
  fifo3/6(fifo_empty) -> Terminator5/1
  [hdr_0x3101] -> bus_create3/1(in1)
  [pol1_id] -> bus_create3/2(in2)
  [hdr_0x3101] -> bus_create2/1(in1)
  [pol1_id] -> bus_create2/2(in2)
  [speadtime0] -> spead_pack2/4(hdr_heap_id), spead_pack2/8(hdr5_0x1600_DIR)  "timein0"
  bus_create3/1(bus_out) -> spead_pack2/9(hdr6_0x3101_DIR)
  [status2] -> spead_pack2/10(hdr7_0x3102_DIR)
  bus_create2/1(bus_out) -> spead_pack3/9(hdr6_0x3101_DIR)
  [status3] -> spead_pack3/10(hdr7_0x3102_DIR)
  [speadtime1] -> spead_pack3/8(hdr5_0x1600_DIR), spead_pack3/4(hdr_heap_id)  "timein1"
  pack_80_64_2/1(ready64) -> pipeline118/1(d)  "r64_00"
  pack_80_64_2/2(valid64) -> Gateway Out82/1, pipeline119/1(d)  "v64_00"
  pack_80_64_2/3(data64) -> pipeline120/1(d)  "d64_00"
  [spead_heapsize] -> spead_pack2/5(hdr_heap_size)
  [spead_heapoffset] -> spead_pack2/6(hdr_heap_offset)
  [spead_pktlen] -> spead_pack2/7(hdr_pkt_len_words)
  [spead_heapsize] -> spead_pack3/5(hdr_heap_size)
  [spead_heapoffset] -> spead_pack3/6(hdr_heap_offset)
  [spead_pktlen] -> spead_pack3/7(hdr_pkt_len_words)
  spead_pack3/4(data_overflow) -> Terminator2/1
  [adc_data_offset] -> spead_pack2/11(hdr8_0x3300)
  [adc_data_offset] -> spead_pack3/11(hdr8_0x3300)
  spead_pack2/4(data_overflow) -> Terminator1/1
  spead_pack2/3(eof) -> pipeline62/1(d)
  spead_pack2/1(data_out) -> pipeline60/1(d)  "packd"
  spead_pack2/2(valid_out) -> pipeline61/1(d)  "packv"
  spead_pack3/1(data_out) -> pipeline63/1(d)
  spead_pack3/2(valid_out) -> pipeline64/1(d)
  spead_pack3/3(eof) -> pipeline65/1(d)
  Inverter1/1 -> fifo3/2(fifo_we_en)
  [tvg_select1] -> Delay106/1
  Mux1/1 -> Assert1/1  "d80_0"
  [data_80_1] -> Delay109/1
  [tvg_pol1] -> Delay108/1
  Assert1/1 -> fifo2/1(data80), bus_expand6/1(bus_in), fifo3/1(data80)
  [fifoselect] -> Gateway Out92/1, Inverter1/1, fifo2/2(fifo_we_en)
  pipeline21/1(q) -> edge_detect12/1(in)
  pipeline22/1(q) -> edge_detect11/1(in)
  pipeline23/1(q) -> [sample_start]
  pipeline24/1(q) -> [sample_end]
  Delay42/1 -> [start_time]
  Delay43/1 -> [end_time]
  Delay49/1 -> [flag_start_time]
  Delay50/1 -> [flag_end_time]
  pipeline10/1(q) -> [gbe_ip3]
  pipeline11/1(q) -> [gbe_ip2]
  pipeline13/1(q) -> [gbe_ip0]
  Delay102/1 -> Gateway Out27/1, Mux/1
  Delay103/1 -> Mux/2
  Delay104/1 -> Mux/3
  Delay106/1 -> Gateway Out23/1, Mux1/1
  Delay126/1 -> [data_enable]
  Delay127/1 -> [sample_mask]
  Delay128/1 -> Gateway Out94/1, tvg_spead_time_with_pkt_ctr/1(localtime64)
  Delay129/1 -> Gateway Out95/1, tvg_spead_time_with_pkt_ctr/2(data_enable)
  Delay130/1 -> Gateway Out96/1, tvg_spead_time_with_pkt_ctr/3(data_mask)
  Delay131/1 -> [tvg_ltime]
  Delay132/1 -> [tvg_stime]
  Delay133/1 -> [tvg_pol0]
  Delay134/1 -> [tvg_pol1]
  [tvg_pol0] -> Delay103/1
  [data_80_0] -> Delay104/1
  Delay109/1 -> Mux1/3
  Delay108/1 -> Mux1/2
  pipeline25/1(q) -> Concat/1
  pipeline26/1(q) -> Concat/2
  pipeline27/1(q) -> Concat1/1
  pipeline28/1(q) -> Concat1/2
  pipeline29/1(q) -> [hdr_0x3101]
  pipeline30/1(q) -> [pol0_id]
  pipeline31/1(q) -> [pol1_id]
  pipeline/1(q) -> edge_detect3/1(in)
  control/2(in_tvg_select0) -> pipeline1/1(d)
  control/3(in_tvg_select1) -> pipeline2/1(d)
  control/4(in_clr_status) -> pipeline3/1(d)
  control/5(in_gbe_rst) -> pipeline4/1(d)
  control/6(in_gbe_txen) -> pipeline5/1(d)
  control/7(in_msync) -> pipeline6/1(d)
  control/8(in_mrst) -> pipeline7/1(d)
  control/9(in_load_tick_offset) -> pipeline8/1(d)
  pipeline8/1(q) -> edge_detect10/1(in)
  pipeline7/1(q) -> edge_detect2/1(in)
  pipeline6/1(q) -> edge_detect1/1(in)
  pipeline4/1(q) -> [gbe_rst]
  pipeline3/1(q) -> edge_detect4/1(in)
  pipeline2/1(q) -> [tvg_select1]
  pipeline1/1(q) -> [tvg_select0]
  pipeline12/1(q) -> [gbe_ip1]
  gbe_iptx0/1(in_reg) -> pipeline13/1(d)
  gbe_iptx1/1(in_reg) -> pipeline12/1(d)
  gbe_iptx2/1(in_reg) -> pipeline11/1(d)
  gbe_iptx3/1(in_reg) -> pipeline10/1(d)
  tick_offset_msw/1(in_reg) -> pipeline17/1(d)
  pipeline17/1(q) -> Concat2/1
  tick_offset_lsw/1(in_reg) -> pipeline18/1(d)
  pipeline18/1(q) -> Concat2/2
  slice1/1 -> pipeline20/1(d)
  pipeline20/1(q) -> local_time_lsw/1(out_reg)
  slice2/1 -> pipeline19/1(d)
  pipeline19/1(q) -> local_time_msw/1(out_reg)
  end_time_lsw/1(in_reg) -> pipeline28/1(d)
  end_time_msw/1(in_reg) -> pipeline27/1(d)
  start_time_lsw/1(in_reg) -> pipeline26/1(d)
  start_time_msw/1(in_reg) -> pipeline25/1(d)
  control_output/4(in_sample_end) -> pipeline24/1(d)
  control_output/3(in_sample_start) -> pipeline23/1(d)
  control_output/2(in_reset_en_time) -> pipeline22/1(d)
  control_output/1(in_load_en_time) -> pipeline21/1(d)
  bus_create/1(bus_out) -> pipeline29/1(d)
  receptor_id/2(in_pol0_id) -> pipeline30/1(d)
  receptor_id/3(in_pol1_id) -> pipeline31/1(d)
  flag_setup/1(in_adc_count) -> pipeline32/1(d)
  flag_setup/2(in_adc_flag) -> pipeline33/1(d)
  flag_setup/3(in_ndiode_flag) -> pipeline34/1(d)
  flag_setup/4(in_load_flags) -> pipeline35/1(d)
  flag_setup/5(in_reset_flags) -> pipeline36/1(d)
  pipeline36/1(q) -> edge_detect8/1(in)
  pipeline35/1(q) -> edge_detect9/1(in)
  pipeline34/1(q) -> [ndiode_flag]
  pipeline33/1(q) -> [adc_flag]
  pipeline32/1(q) -> [adc_count]
  start_flag_msw/1(in_reg) -> pipeline37/1(d)
  pipeline37/1(q) -> Concat4/1
  start_flag_lsw/1(in_reg) -> pipeline38/1(d)
  pipeline38/1(q) -> Concat4/2
  end_flag_msw/1(in_reg) -> pipeline39/1(d)
  pipeline39/1(q) -> Concat5/1
  end_flag_lsw/1(in_reg) -> pipeline40/1(d)
  pipeline40/1(q) -> Concat5/2
  pipeline54/1(q) -> [spead_data0]  "sp0_data"
  pipeline55/1(q) -> [spead_valid0]  "sp0_valid"
  pipeline56/1(q) -> [spead_eof0]  "sp0_eof"
  pipeline57/1(q) -> [spead_data1]  "sp1_data"
  pipeline58/1(q) -> [spead_valid1]  "sp1_valid"
  pipeline59/1(q) -> [spead_eof1]  "sp1_eof"
  pipeline60/1(q) -> [spead_data2]  "sp2_data"
  pipeline61/1(q) -> [spead_valid2]  "sp2_valid"
  pipeline62/1(q) -> [spead_eof2]  "sp2_eof"
  pipeline63/1(q) -> [spead_data3]  "sp3_data"
  pipeline64/1(q) -> [spead_valid3]  "sp3_valid"
  pipeline65/1(q) -> [spead_eof3]  "sp3_eof"
  pipeline97/1(q) -> Gateway Out70/1, pack_80_64_00/2(valid80)
  pipeline98/1(q) -> Gateway Out71/1, pack_80_64_00/3(word_start)
  pipeline99/1(q) -> Logical18/2, Gateway Out72/1, pack_80_64_00/4(pkt_start)
  pipeline101/1(q) -> Gateway Out73/1, pack_80_64_1/2(valid80)
  pipeline102/1(q) -> Gateway Out74/1, pack_80_64_1/3(word_start)
  pipeline105/1(q) -> Gateway Out76/1, pack_80_64_2/2(valid80)
  pipeline106/1(q) -> Gateway Out77/1, pack_80_64_2/3(word_start)
  pipeline109/1(q) -> Gateway Out79/1, pack_80_64_3/2(valid80)
  pipeline110/1(q) -> Gateway Out80/1, pack_80_64_3/3(word_start)
  pipeline112/1(q) -> Logical42/2, [rdy0], Gateway Out26/1
  pipeline113/1(q) -> Logical43/1, Gateway Out69/1, [vld0], Gateway Out25/1
  pipeline115/1(q) -> Logical11/2, [rdy1]
  pipeline116/1(q) -> Logical41/2, [vld1]
  pipeline118/1(q) -> Logical44/2, [rdy2]
  pipeline119/1(q) -> Logical45/1, [vld2]
  pipeline121/1(q) -> Logical46/2, [rdy3]
  pipeline122/1(q) -> Logical47/1, [vld3]
  Delay13/1 -> Logical8/1, Logical6/1
  Delay14/1 -> Logical7/2
  Delay15/1 -> Delay18/1
  Delay16/1 -> Delay19/1
  Delay17/1 -> Logical5/1
  Delay18/1 -> Delay20/1
  Delay19/1 -> Delay21/1
  Delay20/1 -> sample_masking/3(first_samples)
  Delay21/1 -> sample_masking/4(last_samples)
  Delay22/1 -> Logical3/2
  Delay23/1 -> Logical1/1
  Delay24/1 -> Delay25/1
  Delay25/1 -> Delay26/1
  Delay26/1 -> Delay27/1
  Delay27/1 -> sample_masking/1(timei)
  sample_masking/4(flag_valid) -> Delay28/1
  Delay28/1 -> [flag_en]
  Logical1/1 -> sample_masking/7(flag_en)  "flag_en"
  sample_masking/1(timeo) -> Delay29/1
  Delay29/1 -> [masked_time]
  [local_time] -> Delay30/1
  [en_armed] -> Delay31/1
  [local_time] -> Delay32/1, Delay34/1, Delay38/1, Delay40/1
  [start_time] -> Delay33/1
  [end_time] -> Delay35/1, Delay36/1
  Delay30/1 -> Delay24/1
  Delay31/1 -> Delay13/1
  Delay32/1 -> Relational3/1
  Delay33/1 -> Relational3/2
  Delay34/1 -> Relational4/1
  Delay35/1 -> Relational4/2
  Delay36/1 -> Relational5/1
  Delay37/1 -> Relational5/2
  Delay38/1 -> Relational6/1
  Delay39/1 -> Relational6/2
  Delay40/1 -> Relational7/1
  Delay41/1 -> Relational7/2
  Delay44/1 -> Logical4/1, Logical2/1
  Delay45/1 -> Relational/1
  Delay46/1 -> Relational/2
  Delay47/1 -> Relational1/1
  Delay48/1 -> Relational1/2
  Delay51/1 -> Relational2/1
  pipeline127/1(q) -> [pol0_always_on]
  [pol0_always_on] -> gbe0_traffic_control/1(always_on)
  [pol0_requested_pkts] -> gbe0_traffic_control/2(requested_pkts)
  [pol0_offset_data] -> gbe0_traffic_control/3(offset_data)
  [mrst] -> gbe0_traffic_control/4(mrst)
  [pol0_traffic_trigger] -> gbe0_traffic_control/5(traffic_trigger)
  gbe0_traffic_control/1(gbe_txen_gate) -> [gbe_txen_gate0]
  Constant68/1 -> pol1_sample_offset/1(sim_1)
  pipeline129/1(q) -> [pol1_offset_data]
  Constant67/1 -> pol0_sample_offset/1(sim_1)
  pipeline128/1(q) -> [pol0_offset_data]
  Constant69/1 -> pol0_num_pkts/1(sim_1)
  pipeline126/1(q) -> [pol0_requested_pkts]
  Constant73/1 -> pol1_num_pkts/1(sim_1)
  pipeline134/1(q) -> [pol1_requested_pkts]
  pipeline136/1(q) -> [pol1_always_on]
  pipeline5/1(q) -> [gbe_txen]
  Delay/1 -> pol_traffic_trigger/1(sim_1)
  Constant66/1 -> pol_tx_always_on/1(sim_1)
  Constant77/1 -> pol_tx_always_on/2(sim_2)
  pol0_num_pkts/1(in_pol0_num_pkts) -> pipeline126/1(d)
  pol1_num_pkts/1(in_pol1_num_pkts) -> pipeline134/1(d)
  pol_tx_always_on/1(in_pol0_tx_always_on) -> pipeline127/1(d)
  pol_tx_always_on/2(in_pol1_tx_always_on) -> pipeline136/1(d)
  pol0_sample_offset/1(in_pol0_sample_offset) -> pipeline128/1(d)
  pol1_sample_offset/1(in_pol1_sample_offset) -> pipeline129/1(d)
  Delay52/1 -> pol_traffic_trigger/2(sim_2)
  pol_traffic_trigger/1(in_pol0_tx_trigger) -> pipeline131/1(d)
  pipeline130/1(q) -> [pol1_traffic_trigger]
  pol_traffic_trigger/2(in_pol1_tx_trigger) -> pipeline130/1(d)
  edge_detect3/1(out) -> [cnt_rst]  "mrst"
  AddSub/1 -> Slice/1
  AddSub1/1 -> Slice1/1
  [tvg_stime] -> AddSub1/1, AddSub/1
  Constant81/1 -> speadtime0_offset/1(sim_1)
  Slice/1 -> Register5/1
  Slice1/1 -> Register6/1
  speadtime0_offset/1(in_speadtime_offset0) -> AddSub/2
  Constant82/1 -> speadtime1_offset/1(sim_1)
  speadtime1_offset/1(in_speadtime_offset1) -> AddSub1/2
  pipeline131/1(q) -> [pol0_traffic_trigger]
  gbe1_traffic_control/1(gbe_txen_gate) -> [gbe_txen_gate1]
  gbe2_traffic_control/1(gbe_txen_gate) -> [gbe_txen_gate2]
  gbe3_traffic_control/1(gbe_txen_gate) -> [gbe_txen_gate3]
  [spead_valid0] -> gbe0_traffic_control/6(spead_valid)
  [pol0_always_on] -> gbe1_traffic_control/1(always_on)
  [pol0_requested_pkts] -> gbe1_traffic_control/2(requested_pkts)
  [pol0_offset_data] -> gbe1_traffic_control/3(offset_data)
  [mrst] -> gbe1_traffic_control/4(mrst)
  [pol0_traffic_trigger] -> gbe1_traffic_control/5(traffic_trigger)
  [pol1_always_on] -> gbe2_traffic_control/1(always_on)
  [pol1_requested_pkts] -> gbe2_traffic_control/2(requested_pkts)
  [pol1_offset_data] -> gbe2_traffic_control/3(offset_data)
  [mrst] -> gbe2_traffic_control/4(mrst)
  [pol1_traffic_trigger] -> gbe2_traffic_control/5(traffic_trigger)
  [pol1_always_on] -> gbe3_traffic_control/1(always_on)
  [pol1_requested_pkts] -> gbe3_traffic_control/2(requested_pkts)
  [pol1_offset_data] -> gbe3_traffic_control/3(offset_data)
  [mrst] -> gbe3_traffic_control/4(mrst)
  [pol1_traffic_trigger] -> gbe3_traffic_control/5(traffic_trigger)
  [spead_valid1] -> gbe1_traffic_control/6(spead_valid)
  [spead_valid2] -> gbe2_traffic_control/6(spead_valid)
  [spead_valid3] -> gbe3_traffic_control/6(spead_valid)
  Constant59/1 -> Delay/1
  Constant40/1 -> Delay52/1
  master_reset_sim7/1 -> dram_addr_offset/1(sim_1)
  master_reset_sim8/1 -> arb_rst/1(sim_1)
  master_reset_sim9/1 -> arb_en/1(sim_1)
  pipeline133/1(q) -> [arb_en0]
  pipeline138/1(q) -> [dram_addr_offset0]
  master_reset_sim1/1 -> dram_read_length/1(sim_1)
  master_reset_sim2/1 -> dram_rd_trigger/1(sim_1)
  pipeline150/1(q) -> [dram_rd_trig0]
  master_reset_sim3/1 -> dram_tvg/1(sim_1)
  master_reset_sim4/1 -> dram_tvg_length/1(sim_1)
  pipeline148/1(q) -> [dram_tvg_length0]
  edge_detect13/1(out) -> [arb_rst0]
  pipeline135/1(q) -> edge_detect13/1(in)
  master_reset_sim5/1 -> dram_rd_repeat/1(sim_1)
  pipeline151/1(q) -> [dram_rd_repeat0]
  pipeline146/1(q) -> Slice13/1, Slice11/1
  Slice13/1 -> Logical17/1, [tvg_sel0]
  Slice11/1 -> Logical17/2
  Logical17/1 -> [dram_tvg0]
  pipeline149/1(q) -> [dram_read_length0]
  master_reset_sim6/1 -> dram_rd_repeat_rate/1(sim_1)
  pipeline137/1(q) -> [dram_rd_repeat_delay0]
  [cwg_80_0] -> pipeline190/1(d)
  pipeline158/1(q) -> [source_sel_0]
  pipeline159/1(q) -> [source_sel_1]
  Constant87/1 -> src_sel_cntrl/1(sim_1)
  Constant88/1 -> src_sel_cntrl/2(sim_2)
  src_sel_cntrl/1(in_src_sel_0) -> pipeline158/1(d)
  src_sel_cntrl/2(in_src_sel_1) -> pipeline159/1(d)
  [source_sel_0] -> pipeline189/1(d)
  Inverter/1 -> fifo1/2(fifo_we_en)
  Gateway Out24/1 -> To Workspace24/1
  Slice23/1 -> Gateway Out24/1
  Gateway Out25/1 -> To Workspace25/1
  Gateway Out26/1 -> To Workspace26/1
  dram_rd_repeat_rate/1(in_dram_rd_repeat_rate) -> pipeline137/1(d)
  dram_rd_repeat/1(in_dram_rd_repeat) -> pipeline151/1(d)
  dram_tvg/1(in_arb_tvg) -> pipeline146/1(d)
  dram_tvg_length/1(in_tvg_length) -> pipeline148/1(d)
  dram_addr_offset/1(in_dram_addr_offset) -> pipeline138/1(d)
  dram_read_length/1(in_dram_read_length) -> pipeline149/1(d)
  dram_rd_trigger/1(in_arb_trig) -> pipeline150/1(d)
  arb_en/1(in_arb_en) -> pipeline133/1(d)
  arb_rst/1(in_rst) -> pipeline135/1(d)
  pipeline189/1(q) -> Mux5/1
  pipeline190/1(q) -> Mux5/2
  pipeline191/1(q) -> Mux5/3
  [adc_count] -> Concat6/1
  Constant90/1 -> Concat6/2
  Delay4/1 -> [status0]
  Delay55/1 -> [status3]
  Delay54/1 -> [status2]
  Delay53/1 -> [status1]
  Concat6/1 -> Delay55/1, Delay4/1, Delay53/1, Delay54/1
  [ndiode_flag] -> Convert28/1
  Logical/1 -> Convert27/1
  Logical19/1 -> Convert30/1
  [adc_flag] -> Convert29/1
  [flag_en] -> Logical/1, Logical19/2
  Convert28/1 -> Logical/2
  Convert29/1 -> Logical19/1
  Convert30/1 -> Concat6/3
  Convert27/1 -> Concat6/4
  Gateway Out13/1 -> To Workspace13/1
  [local_time] -> pipeline203/1(d)
  [mrst] -> pipeline201/1(d)
  [wng_man_rst0] -> pipeline199/1(d)
  wng_rst/1(wng_rst) -> Gateway Out13/1, [wng_rst0]
  Constant89/1 -> rpt_length_wng0/1(sim_1)
  pipeline200/1(q) -> wng_rst/5(num_samples_for_rst)
  pipeline199/1(q) -> wng_rst/4(man_rst)
  pipeline201/1(q) -> wng_rst/3(mrst)
  pipeline202/1(q) -> wng_rst/2(future_time)
  pipeline203/1(q) -> wng_rst/1(local_time)
  Constant95/1 -> rpt_load_time_msw_wng0/1(sim_1)
  Constant93/1 -> rpt_load_time_lsw_wng0/1(sim_1)
  Concat3/1 -> Delay1/1
  pipeline204/1(q) -> Concat3/1
  pipeline205/1(q) -> Concat3/2
  rpt_load_time_lsw_wng0/1(in_reg) -> pipeline205/1(d)
  rpt_load_time_msw_wng0/1(in_reg) -> pipeline204/1(d)
  Delay1/1 -> pipeline202/1(d)
  rpt_length_wng0/1(in_samples) -> pipeline206/1(d)
  pipeline206/1(q) -> pipeline200/1(d)
  [local_time] -> pipeline154/1(d)
  impulse/1(impulse0) -> [impulse_gen0]
  pipeline152/1(q) -> impulse/2(future_time)
  pipeline154/1(q) -> impulse/1(local_time)
  Constant92/1 -> impulse_load_time_msw/1(sim_1)
  Constant91/1 -> impulse_load_time_lsw/1(sim_1)
  Concat7/1 -> Delay10/1
  pipeline155/1(q) -> Concat7/1
  pipeline160/1(q) -> Concat7/2
  impulse_load_time_lsw/1(in_reg) -> pipeline160/1(d)
  impulse_load_time_msw/1(in_reg) -> pipeline155/1(d)
  Delay10/1 -> pipeline152/1(d)
  pipeline163/1(q) -> Mux5/4
  [impulse_gen0] -> pipeline163/1(d)
  gpio/1 -> Terminator62/1
  Gateway Out/1 -> To Workspace/1
  impulse/2(impulse_gpio) -> [impulse_gpio]
  pipeline145/1(q) -> impulse/3(delay_correction)
  impulse_delay_correction/1(in_reg) -> pipeline145/1(d)
  Constant55/1 -> impulse_delay_correction/1(sim_1)
  pipeline144/1(q) -> Gateway Out/1, gpio/1
  [impulse_gpio] -> pipeline144/1(d)
  bus_create4/1(bus_out) -> pipeline191/1(d)
  [tvg_ltime] -> Delay11/1
  Delay11/1 -> Delay12/1
  [data_80_0] -> Delay56/1
  Delay56/1 -> Delay57/1
  bus_expand14/7(out2) -> pipeline167/1(d)
  bus_expand14/8(lsb_out1) -> pipeline170/1(d)
  bus_expand14/6(out3) -> pipeline171/1(d)
  bus_expand14/5(out4) -> pipeline172/1(d)
  bus_expand14/4(out5) -> pipeline209/1(d)
  bus_expand14/3(out6) -> pipeline210/1(d)
  bus_expand14/2(out7) -> pipeline211/1(d)
  bus_expand14/1(msb_out8) -> pipeline212/1(d)
  pipeline212/1(q) -> ss_fifo_in/1(in_d0)
  pipeline211/1(q) -> ss_fifo_in/2(in_d1)
  pipeline210/1(q) -> ss_fifo_in/3(in_d2)
  pipeline209/1(q) -> ss_fifo_in/4(in_d3)
  pipeline172/1(q) -> ss_fifo_in/5(in_d4)
  pipeline171/1(q) -> ss_fifo_in/6(in_d5)
  pipeline167/1(q) -> ss_fifo_in/7(in_d6)
  pipeline170/1(q) -> ss_fifo_in/8(in_d7)
  Delay57/1 -> bus_expand14/1(bus_in)
  Delay12/1 -> pipeline215/1(d), Relational8/1
  pipeline215/1(q) -> ss_localtime/1(in_time)
  pipeline213/1(q) -> ss_fifo_in/9(in_gpio_trig)
  Delay58/1 -> Delay59/1
  Delay59/1 -> pipeline213/1(d)
  [impulse_gpio] -> Delay60/1
  Delay60/1 -> Delay58/1
  pipeline214/1(q) -> impulse/4(Impulse_offset)
  Constant109/1 -> impulse_offset/1(sim_1)
  impulse_offset/1(in_reg) -> pipeline214/1(d)
  Constant108/1 -> ss_trig_time_msw/1(sim_1)
  Constant107/1 -> ss_trig_time_lsw/1(sim_1)
  Concat8/1 -> Delay61/1
  pipeline216/1(q) -> Concat8/1
  pipeline217/1(q) -> Concat8/2
  ss_trig_time_lsw/1(in_reg) -> pipeline217/1(d)
  ss_trig_time_msw/1(in_reg) -> pipeline216/1(d)
  Delay61/1 -> Relational8/2
  Relational8/1 -> edge_detect/1
  pipeline218/1(q) -> ss_fifo_in/10(we)
  [fifoselect] -> pipeline219/1(d), pipeline218/1(d)
  pipeline219/1(q) -> ss_localtime/2(we)
  edge_detect/1 -> ss_localtime/3(trig), ss_fifo_in/11(trig)
  Constant111/1 -> start_load_time_msw/1(sim_1)
  Constant110/1 -> start_load_time_lsw/1(sim_1)
  pipeline220/1(q) -> Concat9/1
  pipeline221/1(q) -> Concat9/2
  start_load_time_msw/1(in_reg) -> pipeline220/1(d)
  start_load_time_lsw/1(in_reg) -> pipeline221/1(d)
  Concat9/1 -> Delay62/1
  Constant113/1 -> stop_load_time_msw/1(sim_1)
  Constant112/1 -> stop_load_time_lsw/1(sim_1)
  pipeline222/1(q) -> Concat10/1
  pipeline223/1(q) -> Concat10/2
  stop_load_time_msw/1(in_reg) -> pipeline222/1(d)
  stop_load_time_lsw/1(in_reg) -> pipeline223/1(d)
  Concat10/1 -> Delay63/1
  Delay62/1 -> pipeline225/1(d)
  Delay63/1 -> pipeline224/1(d)
  pipeline225/1(q) -> start_stop_cntrl/1(start_time)
  pipeline224/1(q) -> start_stop_cntrl/2(stop_time)
  [mrst] -> start_stop_cntrl/3(rst)
  start_stop_cntrl/1(start_stop_sel) -> [start_stop_sel]
  pipeline195/1(q) -> Mux3/2
  Mux3/1 -> [data_80_0]
  [start_stop_sel] -> Mux3/1
  Constant115/1 -> Mux3/3
  data_ins/1(data) -> Delay73/1
  debug_control/1(in_reg) -> Slice2/1, Slice10/1
  Constant94/1 -> debug_control/1(sim_1)
  Constant120/1 -> pkt_size0/1(sim_1)
  pkt_size0/1(in_reg) -> Delay67/1, Relational9/1
  pkt_size_calc0/1(en_out) -> Delay69/1
  pkt_size_calc0/2(eof) -> Delay70/1
  data_ins/2(en_out) -> Delay74/1
  data_ins/3(eof_out) -> Delay75/1
  [debug_cnt_rst] -> data_ins/1(rst)
  Slice2/1 -> Delay64/1
  Delay64/1 -> [debug_cnt_rst]
  Gateway Out8/1 -> Scope1/1
  Gateway Out10/1 -> Scope1/2
  Gateway Out11/1 -> Scope1/3
  Gateway Out14/1 -> Scope1/4
  Slice3/1 -> Gateway Out8/1
  Slice4/1 -> Gateway Out10/1
  Logical22/1 -> Counter1/2, Gateway Out7/1
  Counter1/1 -> Delay68/1, Gateway Out2/1
  [debug_cnt_rst] -> Counter1/1
  Delay67/1 -> pkt_size_calc0/2(size)
  Delay68/1 -> Convert10/1
  Delay69/1 -> data_ins/2(en_in)
  Delay70/1 -> data_ins/3(eof_in)
  Delay71/1 -> pkt_size_calc0/3(en_in)
  Delay73/1 -> Slice3/1, Slice4/1
  Delay74/1 -> Gateway Out11/1, Logical22/1
  Delay75/1 -> Gateway Out14/1, Logical22/2
  Slice10/1 -> Delay81/1
  pkt_rate0/1(en) -> Delay83/1, Logical23/3
  Logical23/1 -> Delay71/1
  Delay81/1 -> Logical23/2
  Gateway Out2/1 -> Scope4/1
  Gateway Out7/1 -> Scope4/2
  Counter3/1 -> Delay82/1
  Delay82/1 -> debug_rate/1(out_reg)
  Delay83/1 -> Counter3/1
  Constant119/1 -> Relational9/2
  Relational9/1 -> Logical23/1
  [debug_cnt_rst] -> pkt_size_calc0/1(rst)
  Convert10/1 -> debug_tx_pkt_cnt/1(out_reg)
  [forty_gbe_led_up] -> Delay72/1
  [forty_gbe_led_rx] -> Delay101/1
  [forty_gbe_led_tx] -> Delay110/1
  [forty_gbe_tx_afull] -> Delay107/1
  [forty_gbe_tx_overflow] -> Delay112/1
  [forty_gbe_rx_overrun] -> Delay111/1
  [arb_rst0] -> Terminator9/1
  [arb_en0] -> Terminator10/1
  [dram_rd_repeat0] -> Terminator11/1
  [dram_rd_repeat_delay0] -> Terminator13/1
  [tvg_sel0] -> Terminator14/1
  [dram_tvg0] -> Terminator17/1
  [dram_tvg_length0] -> Terminator19/1
  [dram_addr_offset0] -> Terminator21/1
  [dram_read_length0] -> Terminator22/1
  Delay107/1 -> status0/4(out_tx_afull)
  Delay101/1 -> status0/2(out_led_rx)
  Delay112/1 -> status0/5(out_tx_overflow)
  Delay111/1 -> status0/6(out_rx_overrun)
  Delay110/1 -> status0/3(out_led_tx)
  Delay72/1 -> status0/1(out_led_up)
  pipeline15/1(q) -> [gbe_port]
  Constant26/1 -> [spead_heapsize]
  Constant27/1 -> [spead_pktlen]
  Constant45/1 -> [spead_heapoffset]
  Constant8/1 -> [adc_data_offset]
  [spead_data0] -> pipeline72/1(d)
  [spead_valid0] -> pipeline73/1(d)
  wr_addr0/1 -> Gateway Out63/1, 64_to_256/1  "waddr"
  [spead_valid0] -> Gateway Out19/1, edge_detect27/1(in), edge_detect7/1, pipeline67/1(d)
  Constant116/1 -> 64_to_256/6
  Constant121/1 -> 64_to_256/5
  rd_addr0/1 -> Gateway Out64/1, 64_to_256/4, Relational13/2  "rdaddr"
  edge_detect7/1 -> wr_addr0/1
  pipeline67/1(q) -> wr_addr0/2
  pipeline72/1(q) -> 64_to_256/2
  pipeline73/1(q) -> 64_to_256/3  "dv64_0"
  64_to_256/1 -> Terminator25/1
  edge_detect27/1(out) -> rd_addr0/1, rd_arm/3, rd_arm/1
  Constant131/1 -> Relational13/1
  Relational13/1 -> rd_arm/2  "rd_done"
  rd_arm/1 -> pipeline74/1(d), rd_addr0/2  "rd_en"
  edge_detect17/1(out) -> [sp256_eof0]  "eof256_0"
  [spead_data2] -> pipeline77/1(d)
  [spead_valid2] -> pipeline80/1(d)
  wr_addr2/1 -> 64_to_1/1  "waddr"
  [spead_valid2] -> pipeline76/1(d), edge_detect18/1, edge_detect20/1(in), Gateway Out21/1
  Constant21/1 -> 64_to_1/6
  Constant25/1 -> 64_to_1/5
  rd_addr2/1 -> Relational14/2, 64_to_1/4  "rdaddr"
  edge_detect18/1 -> wr_addr2/1
  pipeline76/1(q) -> wr_addr2/2
  pipeline77/1(q) -> 64_to_1/2
  pipeline80/1(q) -> 64_to_1/3  "dv64_2"
  64_to_1/1 -> Terminator26/1
  edge_detect20/1(out) -> rd_addr2/1
  Constant86/1 -> Relational14/1
  Relational14/1 -> rd_arm2/2  "rd_done"
  rd_arm2/1 -> rd_addr2/2, pipeline81/1(d)  "rd_en"
  pipeline81/1(q) -> edge_detect19/1(in), pipeline82/1(d)  "dv256"
  edge_detect19/1(out) -> [sp256_eof2]  "eof256_2"
  pipeline82/1(q) -> [sp256_dv2]  "dv256_2"
  [sp256_eof0] -> rd_arm2/3, rd_arm2/1
  [spead_data1] -> pipeline84/1(d)
  [spead_valid1] -> pipeline85/1(d)
  wr_addr1/1 -> 64_to_2/1  "waddr"
  [spead_valid1] -> pipeline83/1(d), edge_detect21/1, Gateway Out20/1, edge_detect23/1(in)
  Constant122/1 -> 64_to_2/6
  Constant123/1 -> 64_to_2/5
  rd_addr1/1 -> Relational10/2, 64_to_2/4  "rdaddr"
  edge_detect21/1 -> wr_addr1/1
  pipeline83/1(q) -> wr_addr1/2
  pipeline84/1(q) -> 64_to_2/2
  pipeline85/1(q) -> 64_to_2/3  "dv64_1"
  64_to_2/1 -> Terminator27/1
  edge_detect23/1(out) -> rd_arm1/3, rd_arm1/1, rd_addr1/1
  Constant124/1 -> Relational10/1
  Relational10/1 -> rd_arm1/2  "rd_done"
  rd_arm1/1 -> rd_addr1/2, pipeline86/1(d)  "rd_en"
  pipeline86/1(q) -> edge_detect22/1(in), pipeline124/1(d)  "dv256"
  edge_detect22/1(out) -> [sp256_eof1]  "eof256_1"
  pipeline124/1(q) -> [sp256_dv1]  "dv256_1"
  [spead_data3] -> pipeline132/1(d)
  [spead_valid3] -> pipeline139/1(d)
  wr_addr3/1 -> 64_to_3/1  "waddr"
  [spead_valid3] -> edge_detect26/1(in), Gateway Out22/1, edge_detect24/1, pipeline125/1(d)
  Constant125/1 -> 64_to_3/6
  Constant126/1 -> 64_to_3/5
  rd_addr3/1 -> 64_to_3/4, Relational11/2  "rdaddr"
  edge_detect24/1 -> wr_addr3/1
  pipeline125/1(q) -> wr_addr3/2
  pipeline132/1(q) -> 64_to_3/2
  pipeline139/1(q) -> 64_to_3/3  "dv64_3"
  64_to_3/1 -> Terminator24/1
  edge_detect26/1(out) -> rd_addr3/1
  Constant127/1 -> Relational11/1
  Relational11/1 -> rd_arm3/2  "rd_done"
  rd_arm3/1 -> pipeline140/1(d), rd_addr3/2  "rd_en"
  pipeline140/1(q) -> edge_detect25/1(in), pipeline141/1(d)  "dv256"
  edge_detect25/1(out) -> [sp256_eof3]  "eof256_3"
  pipeline141/1(q) -> [sp256_dv3]  "dv256_3"
  [sp256_eof1] -> rd_arm3/1, rd_arm3/3
  [sp256_dv0] -> Mux2/1
  [sp256_data0] -> Mux2/3
  [sp256_data2] -> Mux2/2
  [sp256_dv1] -> pipeline14/1(d)
  Mux2/1 -> Mux7/2
  [sp256_data1] -> pipeline186/1(d)
  [sp256_dv3] -> pipeline16/1(d)
  Mux7/1 -> Mux8/2
  [sp256_data3] -> pipeline187/1(d)
  Mux8/1 -> pipeline193/1(d)
  pipeline186/1(q) -> Mux7/3
  pipeline187/1(q) -> pipeline188/1(d)
  pipeline188/1(q) -> Mux8/3
  [sp256_dvg0] -> Logical38/1
  [sp256_dvg1] -> Logical38/2
  [sp256_dvg2] -> Logical38/3
  [sp256_dvg3] -> Logical38/4
  Logical38/1 -> pipeline229/1(d)
  pipeline229/1(q) -> pipeline231/1(d)
  pipeline231/1(q) -> pipeline169/1(d)
  [sp256_eofg0] -> Logical10/1
  [sp256_eofg2] -> Logical10/3
  Logical10/1 -> pipeline232/1(d)
  pipeline232/1(q) -> pipeline9/1(d)
  pipeline9/1(q) -> pipeline175/1(d)  "tx_eof"
  [sp256_dv0] -> Mux11/1
  [gbe_ip0] -> Mux11/3
  [gbe_ip2] -> Mux11/2
  [sp256_dv1] -> Mux12/1
  Mux11/1 -> Mux12/2
  [gbe_ip1] -> pipeline207/1(d)
  [sp256_dv3] -> Mux13/1
  Mux12/1 -> Mux13/2
  [gbe_ip3] -> pipeline227/1(d)
  Mux13/1 -> Gateway Out1/1
  pipeline207/1(q) -> Mux12/3
  pipeline227/1(q) -> pipeline228/1(d)
  pipeline228/1(q) -> Mux13/3
  [gbe_txen0] -> Logical12/2
  pipeline75/1(q) -> [sp256_dv0]  "dv256_0"
  [sp256_eof0] -> Logical12/1
  [sp256_dv0] -> Logical13/1
  [gbe_txen0] -> Logical13/2
  Logical13/1 -> Gateway Out65/1, [sp256_dvg0]
  Logical12/1 -> Gateway Out90/1, [sp256_eofg0]
  [gbe_txen1] -> Logical14/2
  [sp256_eof1] -> Logical14/1
  [sp256_dv1] -> Logical15/1
  [gbe_txen1] -> Logical15/2
  Logical15/1 -> Gateway Out66/1, [sp256_dvg1]
  Logical14/1 -> Gateway Out89/1, [sp256_eofg1]
  [gbe_txen2] -> Logical16/2
  [sp256_eof2] -> Logical16/1
  [sp256_dv2] -> Logical25/1
  [gbe_txen2] -> Logical25/2
  Logical25/1 -> Gateway Out67/1, [sp256_dvg2]
  Logical16/1 -> Gateway Out88/1, [sp256_eofg2]
  [gbe_txen3] -> Logical26/2
  [sp256_eof3] -> Logical26/1
  [sp256_dv3] -> Logical27/1
  [gbe_txen3] -> Logical27/2
  Logical27/1 -> Gateway Out68/1, [sp256_dvg3]
  Logical26/1 -> Gateway Out87/1, [sp256_eofg3]
  [sp256_dvg0] -> Logical30/1
  [sp256_dvg1] -> Logical28/1
  Logical28/1 -> Logical30/2
  [sp256_dvg3] -> Logical28/3
  [sp256_dvg2] -> Logical28/2
  [sp256_dvg1] -> Logical31/1
  [sp256_dvg0] -> Logical29/1
  Logical29/1 -> Logical31/2
  [sp256_dvg3] -> Logical29/3
  [sp256_dvg2] -> Logical29/2
  [sp256_dvg2] -> Logical33/1
  [sp256_dvg0] -> Logical32/1
  Logical32/1 -> Logical33/2
  [sp256_dvg3] -> Logical32/3
  [sp256_dvg1] -> Logical32/2
  [sp256_dvg3] -> Logical35/1
  [sp256_dvg0] -> Logical34/1
  Logical34/1 -> Logical35/2
  [sp256_dvg2] -> Logical34/3
  [sp256_dvg1] -> Logical34/2
  Logical30/1 -> Logical36/1
  Logical31/1 -> Logical36/2
  Logical33/1 -> Logical36/3
  Logical35/1 -> Logical36/4
  Logical36/1 -> Counter/2  "gbe_dv_error"
  [clr_status] -> Counter/1
  Counter/1 -> gbe_valid_err/1(out_reg)
  pipeline14/1(q) -> Mux7/1
  pipeline16/1(q) -> pipeline66/1(d)
  pipeline66/1(q) -> Mux8/1
  bus_expand/1(msb_out4) -> Terminator35/1  "tx_d3"
  bus_expand/2(out3) -> Terminator36/1  "tx_d2"
  bus_expand/3(out2) -> Terminator37/1  "tx_d1"
  Constant85/1 -> Relational12/2, Relational12/1
  Relational12/1 -> Inverter3/1
  Inverter3/1 -> Logical37/2
  [sp256_eof] -> Logical37/1
  [clr_status] -> Counter2/1
  Counter2/1 -> gbe_last_value_err/1(out_reg)
  Logical37/1 -> Counter2/2  "last_value_error"
  [sp256_data] -> bus_expand/1(bus_in)
  [sel_munge] -> Mux17/1
  Mux17/1 -> [sp256_data3]
  [sel_munge] -> Mux16/1
  Mux16/1 -> [sp256_data2]
  [sel_munge] -> Mux18/1
  Mux18/1 -> [sp256_data1]
  [sel_munge] -> Mux19/1
  Mux19/1 -> [sp256_data0]
  [gbe_rst] -> pipeline233/1(d)
  Constant18/1 -> forty_gbe/7(rx_ack)
  Constant56/1 -> forty_gbe/8(rx_overrun_ack)
  pipeline239/1(q) -> forty_gbe/9(debug_rst)
  Logical40/1 -> pipeline238/1(d)
  Logical39/1 -> pipeline235/1(d)
  [sp256_data] -> pipeline234/1(d)
  [gbe_port] -> pipeline237/1(d)
  [gbe_txip] -> pipeline236/1(d)
  forty_gbe/1(led_up) -> pipeline178/1(d)
  forty_gbe/2(led_rx) -> pipeline87/1(d)
  forty_gbe/3(led_tx) -> pipeline176/1(d)
  forty_gbe/4(tx_afull) -> pipeline177/1(d)
  forty_gbe/5(tx_overflow) -> pipeline179/1(d)
  forty_gbe/12(rx_overrun) -> pipeline197/1(d)
  forty_gbe/6(rx_data) -> Terminator42/1
  forty_gbe/7(rx_valid) -> Terminator43/1
  forty_gbe/10(rx_end_of_frame) -> Terminator44/1
  forty_gbe/11(rx_bad_frame) -> Terminator45/1
  forty_gbe/8(rx_source_ip) -> Terminator7/1
  forty_gbe/9(rx_source_port) -> Terminator8/1
  pipeline178/1(q) -> [forty_gbe_led_up]
  pipeline87/1(q) -> [forty_gbe_led_rx]
  pipeline176/1(q) -> [forty_gbe_led_tx]
  pipeline177/1(q) -> [forty_gbe_tx_afull]
  pipeline179/1(q) -> [forty_gbe_tx_overflow]
  pipeline197/1(q) -> [forty_gbe_rx_overrun]
  forty_gbe/14(rx_dest_port) -> Terminator40/1
  forty_gbe/13(rx_dest_ip) -> Terminator41/1
  [gbe_txen] -> Logical39/1
  [sp256_dv] -> Logical39/2
  [gbe_txen] -> Logical40/1
  [sp256_eof] -> Logical40/2
  pipeline233/1(q) -> forty_gbe/1(rst)
  pipeline234/1(q) -> forty_gbe/2(tx_data)
  pipeline235/1(q) -> forty_gbe/3(tx_valid)
  pipeline236/1(q) -> forty_gbe/4(tx_dest_ip)
  pipeline237/1(q) -> forty_gbe/5(tx_dest_port)
  pipeline238/1(q) -> forty_gbe/6(tx_end_of_frame)
  [cnt_rst] -> pipeline239/1(d)
  ramp0/1 -> [rampdata0]
  [vld0] -> ramp0/2
  [rdy0] -> ramp0/1
  ramp1/1 -> [rampdata1]
  [vld1] -> ramp1/2
  [rdy1] -> ramp1/1
  [spead_data0] -> spead_snap0/1(in_d64)
  [spead_valid0] -> spead_snap0/2(we)
  [spead_eof0] -> spead_detail/1(in_eof)
  [spead_valid0] -> spead_detail/2(in_we), spead_detail/3(we)
  Logical9/1 -> spead_detail/4(trig), spead_snap0/3(trig)
  [spead_eof0] -> Logical9/2
  [speadsnap_arm] -> Logical9/1
  speadsnap_control/1(in_speadsnap_arm) -> Delay65/1
  Delay65/1 -> [speadsnap_arm]
  ramp2/1 -> [rampdata2]
  [vld2] -> ramp2/2
  [rdy2] -> ramp2/1
  ramp3/1 -> [rampdata3]
  [vld3] -> ramp3/2
  [rdy3] -> ramp3/1
  ramp80/1 -> [ramp79]
  [rst_ramp80] -> ramp80/1
  Delay76/1 -> [sel_ramp80]
  ramp_control/1(in_sel_ramp80) -> Delay76/1
  Delay77/1 -> [rst_ramp80]
  ramp_control/2(in_rst_ramp80) -> Delay77/1
  Delay66/1 -> [sel_munge]
  ramp_control/3(in_sel_munge) -> Delay66/1
  gbe_control/1(in_gbe0) -> [gbe_txen0]
  gbe_control/2(in_gbe1) -> [gbe_txen1]
  gbe_control/3(in_gbe2) -> [gbe_txen2]
  gbe_control/4(in_gbe3) -> [gbe_txen3]
  Constant117/1 -> gbe_control/2(sim_2)
  Constant65/1 -> gbe_control/1(sim_1)
  Constant118/1 -> gbe_control/3(sim_3)
  Constant132/1 -> gbe_control/4(sim_4)
  pipeline68/1(q) -> Mux14/2
  [sel_ramp80] -> Mux14/1
  Mux14/1 -> Slice23/1, Gateway Out107/1, spead_pack0/3(data64)
  pack_80_64_00/3(data64) -> pipeline68/1(d)  "d64_00"
  [sel_ramp80] -> Mux15/1
  Mux15/1 -> Gateway Out108/1, spead_pack1/3(data64)
  [sel_ramp80] -> Mux20/1
  Mux20/1 -> Gateway Out109/1, spead_pack2/3(data64)
  [sel_ramp80] -> Gateway Out113/1, Mux21/1
  [ramp79] -> bus_create4/2(in2)  "d80_0"
  Constant133/1 -> bus_create4/1(in1)
  [rampdata0] -> Mux14/3
  [rampdata1] -> Mux15/3
  pipeline117/1(q) -> Mux15/2
  [rampdata2] -> Mux20/3
  pipeline120/1(q) -> Mux20/2
  [rampdata3] -> Mux21/3
  pipeline123/1(q) -> Mux21/2
  Logical11/1 -> spead_pack1/1(data64_ready)
  Logical41/1 -> spead_pack1/2(data64_valid), Gateway Out62/1
  [gbe_txen_gate1] -> Logical41/1, Logical11/1
  [gbe_txen_gate0] -> Logical43/2, Gateway Out60/1, Logical42/1
  Logical43/1 -> Gateway Out61/1, spead_pack0/2(data64_valid)
  Logical42/1 -> spead_pack0/1(data64_ready)
  [gbe_txen_gate2] -> Logical45/2, Logical44/1
  Logical44/1 -> spead_pack2/1(data64_ready)
  Logical45/1 -> spead_pack2/2(data64_valid), Gateway Out85/1
  [gbe_txen_gate3] -> Logical47/2, Logical46/1
  Logical46/1 -> spead_pack3/1(data64_ready)
  Logical47/1 -> spead_pack3/2(data64_valid), Gateway Out86/1
  bram_munge0/1(Out1) -> Mux19/2
  bram_munge1/1(Out1) -> Mux18/2
  bram_munge2/1(Out1) -> Mux16/2
  bram_munge3/1(Out1) -> Mux17/2
  Delay78/1 -> Mux9/1
  [speadtime0] -> Mux9/3
  pipeline96/1(q) -> Mux9/2
  Mux9/1 -> pack_80_64_00/1(data80)
  Logical18/1 -> Delay78/1
  [sel_insert_time] -> Logical18/1
  [mrst] -> Gateway Out98/1, ticks_since_mrst/1(reset)
  [msync] -> Gateway Out99/1, ticks_since_mrst/2(sync)
  control/1(in_cnt_rst) -> pipeline/1(d)
  ramp_control/4(in_sel_insert_time) -> Delay79/1
  Delay79/1 -> [sel_insert_time]
  pipeline103/1(q) -> Logical48/2, Gateway Out75/1, pack_80_64_1/4(pkt_start)
  Delay80/1 -> Mux10/1
  Logical48/1 -> Delay80/1
  [sel_insert_time] -> Logical48/1
  [speadtime1] -> Mux10/3
  pipeline100/1(q) -> Mux10/2
  Mux10/1 -> pack_80_64_1/1(data80)
  Delay84/1 -> Mux22/1
  Logical49/1 -> Delay84/1
  [sel_insert_time] -> Logical49/1
  Mux22/1 -> pack_80_64_2/1(data80)
  [speadtime0] -> Mux22/3
  pipeline104/1(q) -> Mux22/2
  pipeline111/1(q) -> Logical50/2, Gateway Out81/1, pack_80_64_3/4(pkt_start)
  Delay85/1 -> Mux23/1
  Logical50/1 -> Delay85/1
  [sel_insert_time] -> Logical50/1
  Mux23/1 -> pack_80_64_3/1(data80)
  [speadtime1] -> Mux23/3
  pipeline108/1(q) -> Mux23/2
  [start_stop_sel] -> Counter4/2
  Counter4/1 -> start_stop_ctr/1(out_reg)
  [cnt_rst] -> Counter4/1
  [gbe_txen_gate0] -> Counter5/2
  Counter5/1 -> tx_gate_ctrs/1(out_sp0)
  [cnt_rst] -> Counter6/1, Counter7/1, Counter8/1, Counter5/1
  Counter6/1 -> tx_gate_ctrs/2(out_sp1)
  Counter7/1 -> tx_gate_ctrs/3(out_sp2)
  Counter8/1 -> tx_gate_ctrs/4(out_sp3)
  [gbe_txen_gate3] -> Counter8/2
  [gbe_txen_gate2] -> Counter7/2
  [gbe_txen_gate1] -> Counter6/2
  Mux5/1 -> pipeline195/1(d)
  [cwg_80_1] -> pipeline114/1(d)
  [source_sel_1] -> pipeline71/1(d)
  pipeline71/1(q) -> Mux25/1
  pipeline114/1(q) -> Mux25/2
  pipeline142/1(q) -> Mux25/3
  pipeline70/1(q) -> Mux25/4
  [impulse_gen0] -> pipeline70/1(d)
  bus_create5/1(bus_out) -> pipeline142/1(d)
  pipeline143/1(q) -> Mux6/2
  [start_stop_sel] -> Mux6/1
  Constant20/1 -> Mux6/3
  [ramp79] -> bus_create5/2(in2)  "d80_0"
  Constant24/1 -> bus_create5/1(in1)
  Mux25/1 -> pipeline143/1(d)
  scale_wng1/1(in_scale) -> Gateway Out6/1, pipeline47/1(d)
  scale_wng_corr/1(in_scale) -> pipeline46/1(d)
  [wng0_tp0] -> pipeline91/1(d)
  [wng1_tp0] -> pipeline94/1(d)
  cwg_corr/1(bus_out) -> pipeline90/1(d)
  bus_addsub2/1(dout) -> Delay8/1
  bus_addsub4/1(dout) -> bus_convert6/1(din)
  bus_mult/1(a*b) -> [cwg0_tp1], bus_convert/1(din)
  bus_addsub5/1(dout) -> bus_convert7/1(din)
  bus_mult1/1(a*b) -> bus_convert1/1(din), [cwg1_tp1]
  scale_out1/1(in_scale) -> Gateway Out3/1, pipeline79/1(d)
  Constant1/1 -> scale_wng_corr/1(sim_1)
  pipeline45/1(q) -> [wng_scale0]
  pipeline46/1(q) -> [wng_scale_corr]
  pipeline47/1(q) -> [wng_scale1]
  Delay8/1 -> bus_convert4/1(din)
  Delay139/1 -> bus_addsub4/1(a)
  Delay9/1 -> bus_addsub5/1(a)
  Delay86/1 -> bus_addsub5/2(b)
  pipeline88/1(q) -> bus_mult1/1(a), [cwg1_tp0]
  pipeline79/1(q) -> bus_mult1/2(b)
  pipeline78/1(q) -> bus_mult/2(b)
  pipeline91/1(q) -> bus_addsub/1(a)
  pipeline92/1(q) -> bus_addsub/2(b)
  pipeline93/1(q) -> bus_addsub1/1(a)
  [wng_corr_tp0] -> pipeline93/1(d), pipeline92/1(d)
  pipeline94/1(q) -> bus_addsub1/2(b)
  [cwg_corr] -> bus_addsub2/2(b)
  pipeline156/1(q) -> [cwg_80_0]
  pipeline157/1(q) -> [cwg_80_1]
  Delay5/1 -> bus_addsub4/2(b)
  bus_convert/1(dout) -> [cwg0_tp2], pipeline156/1(d)
  bus_convert2/1(dout) -> [wng_sum0]
  bus_convert3/1(dout) -> [wng_sum1]
  bus_convert4/1(dout) -> [cwg_corr_out0]
  bus_convert5/1(dout) -> [cwg_corr_out1]
  bus_convert6/1(dout) -> pipeline53/1(d)
  bus_convert7/1(dout) -> pipeline88/1(d)
  Constant32/1 -> scale_wng1/1(sim_1)
  scale_wng0/1(in_scale) -> Gateway Out17/1, pipeline45/1(d)
  scale_out0/1(in_scale) -> Gateway Out5/1, pipeline78/1(d)
  Constant64/1 -> freq_cwg0/1(sim_1)
  scale_cwg0/1(in_scale) -> pipeline48/1(d)
  freq_cwg0/1(in_frequency) -> pipeline49/1(d)
  Constant79/1 -> freq_cwg_corr/1(sim_1)
  freq_cwg_corr/1(in_frequency) -> pipeline51/1(d)
  scale_cwg_corr/1(in_scale) -> pipeline50/1(d)
  Constant80/1 -> scale_cwg_corr/1(sim_1)
  Constant58/1 -> scale_out1/1(sim_1)
  Constant57/1 -> scale_out0/1(sim_1)
  pipeline49/1(q) -> cwg0/1(freq)
  pipeline48/1(q) -> cwg0/2(scale)
  [mrst] -> pipeline180/1(d)
  Constant62/1 -> rpt_length_cwg0/1(sim_1)
  rpt_en_cwg0/1(in_en) -> Convert25/1
  Constant70/1 -> rpt_en_cwg0/1(sim_1)
  Convert25/1 -> pipeline181/1(d)
  cwg0/1(bus_out) -> pipeline95/1(d)
  rpt_length_cwg0/1(in_repeat_length) -> pipeline182/1(d)
  pipeline180/1(q) -> cwg0/3(rst)
  pipeline181/1(q) -> cwg0/4(repeat_en)
  pipeline182/1(q) -> cwg0/5(repeat_length)
  cwg0/3(rpt_rst) -> Terminator61/1
  Constant28/1 -> man_rst_wng0/1(sim_1)
  Logical20/1 -> pipeline198/1(d)
  man_rst_wng0/1(in_rst) -> [wng_man_rst0], Logical20/2
  [wng_rst0] -> Logical20/1
  pipeline51/1(q) -> cwg_corr/1(freq)
  pipeline50/1(q) -> cwg_corr/2(scale)
  pipeline147/1(q) -> cwg_corr/3(rst)
  pipeline161/1(q) -> cwg_corr/4(repeat_en)
  pipeline162/1(q) -> cwg_corr/5(repeat_length)
  Constant96/1 -> cwg_corr/6(en)
  [mrst] -> pipeline147/1(d)
  rpt_en_cwg_corr/1(in_en) -> pipeline161/1(d)
  cwg_corr/3(rpt_rst) -> Terminator64/1
  cwg_corr/2(dvalid) -> Terminator65/1
  Constant97/1 -> rpt_en_cwg_corr/1(sim_1)
  rpt_length_cwg_corr/1(in_repeat_length) -> pipeline162/1(d)
  Constant99/1 -> rpt_length_cwg_corr/1(sim_1)
  pipeline53/1(q) -> [cwg0_tp0], bus_mult/1(a)
  pipeline165/1(q) -> wng1/2(rst)
  Logical21/1 -> pipeline165/1(d)
  man_rst_wng1/1(in_rst) -> [wng_man_rst1], Logical21/2
  [wng_rst0] -> Logical21/1
  Constant100/1 -> man_rst_wng1/1(sim_1)
  pipeline166/1(q) -> wng_corr/2(rst)
  Logical24/1 -> pipeline166/1(d)
  man_rst_wng_corr/1(in_rst) -> [wng_man_rst_corr], Logical24/2
  [wng_rst0] -> Logical24/1
  Constant101/1 -> man_rst_wng_corr/1(sim_1)
  Gateway Out3/1 -> To Workspace3/1
  Gateway Out5/1 -> To Workspace5/1
  bus_convert1/1(dout) -> [cwg1_tp2], pipeline157/1(d)
  Gateway Out6/1 -> To Workspace6/1
  Gateway Out17/1 -> To Workspace17/1
  Constant106/1 -> cwg0/6(en)
  pipeline95/1(q) -> [cwg0], bus_expand2/1(bus_in)
  cwg0/2(dvalid) -> Terminator30/1
  [wng_sum0] -> Delay139/1
  [cwg_corr_out0] -> Delay5/1
  [cwg0] -> bus_addsub2/1(a)
  [cwg_corr_out1] -> Delay86/1
  Constant37/1 -> scale_cwg0/1(sim_1)
  Constant36/1 -> freq_cwg1/1(sim_1)
  scale_cwg1/1(in_scale) -> pipeline44/1(d)
  freq_cwg1/1(in_frequency) -> pipeline52/1(d)
  pipeline52/1(q) -> cwg1/1(freq)
  pipeline44/1(q) -> cwg1/2(scale)
  [mrst] -> pipeline41/1(d)
  Constant33/1 -> rpt_length_cwg1/1(sim_1)
  rpt_en_cwg1/1(in_en) -> Convert1/1
  Constant41/1 -> rpt_en_cwg1/1(sim_1)
  Convert1/1 -> pipeline42/1(d)
  cwg1/1(bus_out) -> pipeline89/1(d)
  rpt_length_cwg1/1(in_repeat_length) -> pipeline43/1(d)
  pipeline41/1(q) -> cwg1/3(rst)
  pipeline42/1(q) -> cwg1/4(repeat_en)
  pipeline43/1(q) -> cwg1/5(repeat_length)
  cwg1/3(rpt_rst) -> Terminator29/1
  Constant23/1 -> cwg1/6(en)
  pipeline89/1(q) -> [cwg1]
  cwg1/2(dvalid) -> Terminator28/1
  Constant30/1 -> scale_cwg1/1(sim_1)
  Constant35/1 -> scale_wng0/1(sim_1)
  pipeline90/1(q) -> [cwg_corr]
  [cwg1] -> bus_addsub3/1(a)
  bus_addsub3/1(dout) -> Delay2/1
  Delay2/1 -> bus_convert5/1(din)
  [cwg_corr] -> bus_addsub3/2(b)
  [wng_sum1] -> Delay9/1
  bus_addsub1/1(dout) -> Delay6/1
  Delay6/1 -> bus_convert3/1(din)
  bus_addsub/1(dout) -> Delay7/1
  Delay7/1 -> bus_convert2/1(din)
  Mux6/1 -> [data_80_1]
  [wng_scale0] -> wng0/1(scale_16_14)
  pipeline198/1(q) -> wng0/2(rst)
  wng0/1(bus_out) -> [wng0_tp0]
  [wng_scale1] -> wng1/1(scale_16_14)
  [wng_scale_corr] -> wng_corr/1(scale_16_14)
  wng1/1(bus_out) -> [wng1_tp0]
  wng_corr/1(bus_out) -> [wng_corr_tp0]
  Gateway Out1/1 -> To Workspace1/1
  Gateway Out4/1 -> To Workspace9/1
  Gateway Out9/1 -> To Workspace4/1
  Gateway Out12/1 -> To Workspace7/1
  Gateway Out15/1 -> To Workspace8/1
  bus_expand1/1(msb_out4) -> Gateway Out15/1
  bus_expand1/2(out3) -> Gateway Out4/1
  Gateway Out16/1 -> To Workspace10/1
  bus_expand1/3(out2) -> Gateway Out16/1
  Gateway Out18/1 -> To Workspace38/1
  bus_expand1/4(lsb_out1) -> Gateway Out18/1
  Gateway Out19/1 -> To Workspace11/1
  Gateway Out20/1 -> To Workspace12/1
  Gateway Out21/1 -> To Workspace14/1
  Gateway Out22/1 -> To Workspace15/1
  Gateway Out23/1 -> To Workspace16/1
  Gateway Out27/1 -> To Workspace18/1
  Constant61/1 -> control/2(sim_2)
  Constant44/1 -> control/3(sim_3)
  Constant60/1 -> control/1(sim_1)
  Constant63/1 -> control/4(sim_4)
  Constant71/1 -> control/5(sim_5)
  Constant72/1 -> control/6(sim_6)
  Constant74/1 -> control/7(sim_7)
  Constant75/1 -> control/8(sim_8)
  Constant76/1 -> control/9(sim_9)
  Gateway Out31/1 -> To Workspace30/1
  Gateway Out28/1 -> To Workspace21/1
  Gateway Out29/1 -> To Workspace29/1
  Gateway Out30/1 -> To Workspace28/1
  bus_expand3/1(msb_out8) -> Gateway Out28/1
  bus_expand3/2(out7) -> Gateway Out31/1
  bus_expand3/4(out5) -> Gateway Out30/1
  bus_expand3/3(out6) -> Gateway Out29/1
  bus_expand3/8(lsb_out1) -> Gateway Out34/1
  bus_expand3/7(out2) -> Gateway Out33/1
  bus_expand3/6(out3) -> Gateway Out35/1
  bus_expand3/5(out4) -> Gateway Out32/1
  Gateway Out34/1 -> To Workspace20/1
  Gateway Out33/1 -> To Workspace22/1
  Gateway Out35/1 -> To Workspace23/1
  Gateway Out32/1 -> To Workspace27/1
  [cwg_80_0] -> bus_expand3/1(bus_in)
  Gateway Out39/1 -> To Workspace37/1
  Gateway Out36/1 -> To Workspace31/1
  Gateway Out37/1 -> To Workspace36/1
  Gateway Out38/1 -> To Workspace35/1
  bus_expand4/1(msb_out8) -> Gateway Out36/1
  bus_expand4/2(out7) -> Gateway Out39/1
  bus_expand4/4(out5) -> Gateway Out38/1
  bus_expand4/3(out6) -> Gateway Out37/1
  bus_expand4/8(lsb_out1) -> Gateway Out42/1
  bus_expand4/7(out2) -> Gateway Out41/1
  bus_expand4/6(out3) -> Gateway Out43/1
  bus_expand4/5(out4) -> Gateway Out40/1
  Gateway Out42/1 -> To Workspace19/1
  Gateway Out41/1 -> To Workspace32/1
  Gateway Out43/1 -> To Workspace33/1
  Gateway Out40/1 -> To Workspace34/1
  [cwg_80_1] -> bus_expand4/1(bus_in)
  Gateway Out47/1 -> To Workspace46/1
  Gateway Out44/1 -> To Workspace39/1
  Gateway Out45/1 -> To Workspace45/1
  Gateway Out46/1 -> To Workspace44/1
  bus_expand5/1(msb_out8) -> Gateway Out44/1
  bus_expand5/2(out7) -> Gateway Out47/1
  bus_expand5/4(out5) -> Gateway Out46/1
  bus_expand5/3(out6) -> Gateway Out45/1
  bus_expand5/8(lsb_out1) -> Gateway Out50/1
  bus_expand5/7(out2) -> Gateway Out49/1
  bus_expand5/6(out3) -> Gateway Out51/1
  bus_expand5/5(out4) -> Gateway Out48/1
  Gateway Out50/1 -> To Workspace40/1
  Gateway Out49/1 -> To Workspace41/1
  Gateway Out51/1 -> To Workspace42/1
  Gateway Out48/1 -> To Workspace43/1
  bus_expand6/1(msb_out8) -> Gateway Out52/1
  bus_expand6/2(out7) -> Gateway Out55/1
  bus_expand6/4(out5) -> Gateway Out54/1
  bus_expand6/3(out6) -> Gateway Out53/1
  bus_expand6/8(lsb_out1) -> Gateway Out58/1
  bus_expand6/7(out2) -> Gateway Out57/1
  bus_expand6/6(out3) -> Gateway Out59/1
  bus_expand6/5(out4) -> Gateway Out56/1
  Gateway Out58/1 -> To Workspace47/1
  Gateway Out57/1 -> To Workspace48/1
  Gateway Out59/1 -> To Workspace49/1
  Gateway Out56/1 -> To Workspace50/1
  Gateway Out54/1 -> To Workspace51/1
  Gateway Out55/1 -> To Workspace53/1
  Gateway Out53/1 -> To Workspace52/1
  Gateway Out52/1 -> To Workspace54/1
  bus_expand/4(lsb_out1) -> Terminator31/1  "tx_d0"
  Gateway Out60/1 -> To Workspace2/1
  Gateway Out61/1 -> To Workspace55/1
  Gateway Out62/1 -> To Workspace56/1
  Gateway Out63/1 -> To Workspace57/1
  Gateway Out64/1 -> To Workspace58/1
  Gateway Out65/1 -> To Workspace59/1
  Gateway Out66/1 -> To Workspace60/1
  Gateway Out67/1 -> To Workspace61/1
  Gateway Out68/1 -> To Workspace62/1
  Gateway Out69/1 -> To Workspace63/1
  Gateway Out70/1 -> To Workspace64/1
  Gateway Out71/1 -> To Workspace65/1
  Gateway Out72/1 -> To Workspace66/1
  Gateway Out73/1 -> To Workspace67/1
  Gateway Out74/1 -> To Workspace68/1
  Gateway Out75/1 -> To Workspace69/1
  Gateway Out76/1 -> To Workspace70/1
  Gateway Out77/1 -> To Workspace71/1
  Gateway Out78/1 -> To Workspace72/1
  pipeline107/1(q) -> Logical49/2, Gateway Out78/1, pack_80_64_2/4(pkt_start)
  Gateway Out79/1 -> To Workspace73/1
  Gateway Out80/1 -> To Workspace74/1
  Gateway Out81/1 -> To Workspace75/1
  Gateway Out82/1 -> To Workspace76/1
  Gateway Out83/1 -> To Workspace77/1
  Gateway Out84/1 -> To Workspace78/1
  Gateway Out85/1 -> To Workspace79/1
  Gateway Out86/1 -> To Workspace80/1
  Gateway Out87/1 -> To Workspace81/1
  Gateway Out88/1 -> To Workspace82/1
  Gateway Out89/1 -> To Workspace83/1
  Gateway Out90/1 -> To Workspace84/1
  Gateway Out91/1 -> To Workspace85/1
  Gateway Out92/1 -> To Workspace86/1
